simulink model "Manu6DOF_MICO_NE_v6articulation2019b"  (R2019b)
settings: Solver=ode5  StartTime=0.0  StopTime=10.0  FixedStep=0.001  RelTol=1e-3
undefined symbols (not defined in the file): f, Sub02MIHM
libraries: instrumentlib x27, dspnetwork x24, simulink x7, dspmtrx3 x3, dspsrcs4 x1
(part 2 of 3)

== matlab function Manu6DOF_MICO_NE_v6articulation2019b/C1 ==
  data: qm input; C output; dqm input
function C = fcn(qm, dqm)

% theta_1 = qm(1);
% theta_2 = qm(2);
% theta_3 = qm(3);
% theta_4 = qm(4);
% theta_5 = qm(5);
% theta_6 = qm(6);

q1 = qm(1);
q2 = qm(2);
q3 = qm(3);
q4 = qm(4);
q5 = qm(5);
q6 = qm(6);

q1d = dqm(1);
q2d = dqm(2);
q3d = dqm(3);
q4d = dqm(4);
q5d = dqm(5);
q6d = dqm(6);

%%%%%%%%%%%%%%%%%%%%%%%
%function C_c = Cq(q1,q2,q3,q4,q5,q6,q1d,q2d,q3d,q4d,q5d,q6d)
%CQ
%    C_C = CQ(Q1,Q2,Q3,Q4,Q5,Q6,Q1D,Q2D,Q3D,Q4D,Q5D,Q6D)

%    This function was generated by the Symbolic Math Toolbox version 8.4.
%    09-Jul-2020 20:13:25

C = reshape([q1d.*(-2.356599459063229e+4)-q2d.*4.088711718154727e+4+q3d.*2.730577954033007e+5+q4d.*8.285703356363623e+4-q5d.*1.473618543709382e+5+q6d.*7.520537517824024e+4+sqrt(3.0).*q1d.*1.522529520000002e+4+sqrt(3.0).*q2d.*1.015019680000001e+4+sqrt(3.0).*q3d.*3.555581400000001e+4+sqrt(3.0).*q4d.*3.525894120000001e+4+sqrt(3.0).*q5d.*3.780719200000012e+3+sqrt(3.0).*q6d.*2.486339999999987e+3+q1d.*conj(q1).*5.04570275175e+3+q1d.*conj(q2).*4.49975074899e+3+q2d.*conj(q1).*1.49991691633e+3+q1d.*conj(q3).*1.97644016599907e-13+q2d.*conj(q2).*2.99983383266e+3+q3d.*conj(q1).*6.588133886663567e-14+q1d.*conj(q4).*7.944161321388966e-14+q2d.*conj(q3).*1.317626777332713e-13+q3d.*conj(q2).*6.588133886663567e-14+q4d.*conj(q1).*2.648053773796322e-14-q1d.*conj(q5).*7.310773996869955e-14+q2d.*conj(q4).*5.296107547592644e-14+q3d.*conj(q3).*1.07592391394e+3+q4d.*conj(q2).*2.648053773796322e-14-q5d.*conj(q1).*2.436924665623318e-14+q1d.*conj(q6).*2.003216001705283e-13-q2d.*conj(q5).*4.873849331246636e-14+q3d.*conj(q4).*4.3246e+2+q4d.*conj(q3).*4.3246e+2-q5d.*conj(q2).*2.436924665623318e-14+q6d.*conj(q1).*6.677386672350943e-14+q2d.*conj(q6).*1.335477334470189e-13-q3d.*conj(q5).*3.9798e+2+q4d.*conj(q4).*8.6492e+2-q5d.*conj(q3).*3.9798e+2+q6d.*conj(q2).*6.677386672350943e-14+q3d.*conj(q6).*3.635000000000001e+2+q4d.*conj(q5).*3.9798e+2+q5d.*conj(q4).*3.9798e+2+q6d.*conj(q3).*3.635e+2-q4d.*conj(q6).*3.634999999999999e+2+q5d.*conj(q5).*7.9596e+2-q6d.*conj(q4).*3.635e+2-q5d.*conj(q6).*7.269999999999999e+2-q6d.*conj(q5).*7.27e+2+q6d.*conj(q6).*7.270000000000001e+2-sqrt(3.0).*q1d.*conj(q4).*1.29738e+3-sqrt(3.0).*q4d.*conj(q1).*4.3246e+2-sqrt(3.0).*q1d.*conj(q5).*1.19394e+3-sqrt(3.0).*q2d.*conj(q4).*8.6492e+2-sqrt(3.0).*q4d.*conj(q2).*4.3246e+2-sqrt(3.0).*q5d.*conj(q1).*3.9798e+2+sqrt(3.0).*q1d.*conj(q6).*1.0905e+3-sqrt(3.0).*q2d.*conj(q5).*7.9596e+2-sqrt(3.0).*q3d.*conj(q4).*4.3246e+2+sqrt(3.0).*q4d.*conj(q3).*2.902843497617834e-31-sqrt(3.0).*q5d.*conj(q2).*3.9798e+2+sqrt(3.0).*q6d.*conj(q1).*3.635e+2+sqrt(3.0).*q2d.*conj(q6).*7.27e+2-sqrt(3.0).*q3d.*conj(q5).*3.9798e+2-sqrt(3.0).*q4d.*conj(q4).*4.3246e+2+sqrt(3.0).*q5d.*conj(q3).*2.671400025856601e-31+sqrt(3.0).*q6d.*conj(q2).*3.635e+2+sqrt(3.0).*q3d.*conj(q6).*3.635e+2-sqrt(3.0).*q4d.*conj(q5).*3.9798e+2-sqrt(3.0).*q6d.*conj(q3).*4.451591114900629e-14+sqrt(3.0).*q4d.*conj(q6).*3.635e+2-sqrt(3.0).*q5d.*conj(q5).*3.9798e+2-sqrt(3.0).*q6d.*conj(q4).*4.451591114900629e-14+sqrt(3.0).*q5d.*conj(q6).*3.635e+2+sqrt(3.0).*q6d.*conj(q5).*4.879913108190735e-31+sqrt(3.0).*q6d.*conj(q6).*3.635e+2,q1d.*(-4.088711718154727e+4)-q2d.*4.088711718154727e+4+q3d.*1.398366081578192e+5+q4d.*3.824377798181812e+4-q5d.*7.746164638546913e+4+q6d.*4.008902758912012e+4+sqrt(3.0).*q1d.*1.015019680000001e+4+sqrt(3.0).*q2d.*1.015019680000001e+4+sqrt(3.0).*q3d.*3.30182648e+4+sqrt(3.0).*q4d.*3.272139200000001e+4+sqrt(3.0).*q5d.*1.890359600000006e+3+sqrt(3.0).*q6d.*1.243169999999994e+3+q1d.*conj(q1).*1.49991691633e+3+q1d.*conj(q2).*2.99983383266e+3+q2d.*conj(q1).*1.49991691633e+3+q1d.*conj(q3).*1.317626777332713e-13+q2d.*conj(q2).*2.99983383266e+3+q3d.*conj(q1).*3.294066943331783e-14+q1d.*conj(q4).*5.296107547592644e-14+q2d.*conj(q3).*1.317626777332713e-13+q3d.*conj(q2).*6.588133886663567e-14+q4d.*conj(q1).*1.324026886898161e-14-q1d.*conj(q5).*4.873849331246636e-14+q2d.*conj(q4).*5.296107547592644e-14+q3d.*conj(q3).*1.07592391394e+3+q4d.*conj(q2).*2.648053773796322e-14-q5d.*conj(q1).*1.218462332811659e-14+q1d.*conj(q6).*1.335477334470189e-13-q2d.*conj(q5).*4.873849331246636e-14+q3d.*conj(q4).*4.3246e+2+q4d.*conj(q3).*4.3246e+2-q5d.*conj(q2).*2.436924665623318e-14+q6d.*conj(q1).*3.338693336175472e-14+q2d.*conj(q6).*1.335477334470189e-13-q3d.*conj(q5).*3.9798e+2+q4d.*conj(q4).*8.6492e+2-q5d.*conj(q3).*3.9798e+2+q6d.*conj(q2).*6.677386672350943e-14+q3d.*conj(q6).*3.635e+2+q4d.*conj(q5).*3.9798e+2+q5d.*conj(q4).*3.9798e+2+q6d.*conj(q3).*3.635e+2-q4d.*conj(q6).*3.635e+2+q5d.*conj(q5).*7.9596e+2-q6d.*conj(q4).*3.635e+2-q5d.*conj(q6).*7.27e+2-q6d.*conj(q5).*7.27e+2+q6d.*conj(q6).*7.27e+2-sqrt(3.0).*q1d.*conj(q4).*8.6492e+2-sqrt(3.0).*q4d.*conj(q1).*2.1623e+2-sqrt(3.0).*q1d.*conj(q5).*7.9596e+2-sqrt(3.0).*q2d.*conj(q4).*8.6492e+2-sqrt(3.0).*q4d.*conj(q2).*4.3246e+2-sqrt(3.0).*q5d.*conj(q1).*1.9899e+2+sqrt(3.0).*q1d.*conj(q6).*7.27e+2-sqrt(3.0).*q2d.*conj(q5).*7.9596e+2-sqrt(3.0).*q3d.*conj(q4).*2.1623e+2+sqrt(3.0).*q4d.*conj(q3).*2.902843497617834e-31-sqrt(3.0).*q5d.*conj(q2).*3.9798e+2+sqrt(3.0).*q6d.*conj(q1).*1.8175e+2+sqrt(3.0).*q2d.*conj(q6).*7.27e+2-sqrt(3.0).*q3d.*conj(q5).*1.9899e+2-sqrt(3.0).*q4d.*conj(q4).*2.1623e+2+sqrt(3.0).*q5d.*conj(q3).*2.671400025856601e-31+sqrt(3.0).*q6d.*conj(q2).*3.635e+2+sqrt(3.0).*q3d.*conj(q6).*1.8175e+2-sqrt(3.0).*q4d.*conj(q5).*1.9899e+2-sqrt(3.0).*q6d.*conj(q3).*4.451591114900629e-14+sqrt(3.0).*q4d.*conj(q6).*1.8175e+2-sqrt(3.0).*q5d.*conj(q5).*1.9899e+2-sqrt(3.0).*q6d.*conj(q4).*4.451591114900629e-14+sqrt(3.0).*q5d.*conj(q6).*1.8175e+2+sqrt(3.0).*q6d.*conj(q5).*4.879913108190735e-31+sqrt(3.0).*q6d.*conj(q6).*1.8175e+2,q1d.*2.730577954033007e+5+q2d.*1.398366081578192e+5+q3d.*3.095751114833673e+5+q4d.*5.443043298181812e+4-q5d.*6.047936538546912e+4+q6d.*5.627568258912012e+4+sqrt(3.0).*q1d.*3.555581400000001e+4+sqrt(3.0).*q2d.*3.30182648e+4+sqrt(3.0).*q3d.*6.09614312e+4+sqrt(3.0).*q4d.*4.54242006e+4+sqrt(3.0).*q5d.*1.50919214e+4+sqrt(3.0).*q6d.*1.494348499999999e+4+q1d.*conj(q1).*6.588133886663567e-14+q1d.*conj(q2).*6.588133886663567e-14+q2d.*conj(q1).*3.294066943331783e-14+q1d.*conj(q3).*1.07592391394e+3+q2d.*conj(q2).*6.588133886663567e-14+q3d.*conj(q1).*6.588133886663567e-14+q1d.*conj(q4).*4.3246e+2+q2d.*conj(q3).*1.07592391394e+3+q3d.*conj(q2).*6.588133886663567e-14+q4d.*conj(q1).*1.324026886898161e-14-q1d.*conj(q5).*3.9798e+2+q2d.*conj(q4).*4.3246e+2+q3d.*conj(q3).*2.15184782788e+3+q4d.*conj(q2).*1.324026886898161e-14-q5d.*conj(q1).*1.218462332811659e-14+q1d.*conj(q6).*3.635000000000001e+2-q2d.*conj(q5).*3.9798e+2+q3d.*conj(q4).*8.6492e+2+q4d.*conj(q3).*4.3246e+2-q5d.*conj(q2).*1.218462332811659e-14+q6d.*conj(q1).*3.338693336175472e-14+q2d.*conj(q6).*3.635e+2-q3d.*conj(q5).*7.9596e+2+q4d.*conj(q4).*1.08115e+3-q5d.*conj(q3).*3.9798e+2+q6d.*conj(q2).*3.338693336175472e-14+q3d.*conj(q6).*7.27e+2+q4d.*conj(q5).*1.9899e+2+q5d.*conj(q4).*3.9798e+2+q6d.*conj(q3).*3.635e+2-q4d.*conj(q6).*1.8175e+2+q5d.*conj(q5).*5.9697e+2-q6d.*conj(q4).*3.635e+2-q5d.*conj(q6).*5.4525e+2-q6d.*conj(q5).*7.27e+2+q6d.*conj(q6).*9.0875e+2-sqrt(3.0).*q1d.*conj(q4).*4.3246e+2-sqrt(3.0).*q4d.*conj(q1).*2.1623e+2-sqrt(3.0).*q1d.*conj(q5).*3.9798e+2-sqrt(3.0).*q2d.*conj(q4).*2.1623e+2-sqrt(3.0).*q4d.*conj(q2).*2.1623e+2-sqrt(3.0).*q5d.*conj(q1).*1.9899e+2+sqrt(3.0).*q1d.*conj(q6).*3.635e+2-sqrt(3.0).*q2d.*conj(q5).*1.9899e+2+sqrt(3.0).*q3d.*conj(q4).*5.805686995235668e-31+sqrt(3.0).*q4d.*conj(q3).*2.902843497617834e-31-sqrt(3.0).*q5d.*conj(q2).*1.9899e+2+sqrt(3.0).*q6d.*conj(q1).*1.8175e+2+sqrt(3.0).*q2d.*conj(q6).*1.8175e+2+sqrt(3.0).*q3d.*conj(q5).*5.342800051713201e-31+sqrt(3.0).*q4d.*conj(q4).*4.354265246426751e-31+sqrt(3.0).*q5d.*conj(q3).*2.671400025856601e-31+sqrt(3.0).*q6d.*conj(q2).*1.8175e+2-sqrt(3.0).*q3d.*conj(q6).*8.903182229801258e-14+sqrt(3.0).*q4d.*conj(q5).*1.3357000129283e-31-sqrt(3.0).*q6d.*conj(q3).*4.451591114900629e-14-sqrt(3.0).*q4d.*conj(q6).*6.677386672350943e-14-sqrt(3.0).*q5d.*conj(q5).*1.3357000129283e-31-sqrt(3.0).*q6d.*conj(q4).*4.451591114900629e-14-sqrt(3.0).*q5d.*conj(q6).*2.225795557450314e-14+sqrt(3.0).*q6d.*conj(q5).*4.879913108190735e-31-sqrt(3.0).*q6d.*conj(q6).*2.225795557450315e-14,q1d.*8.285703356363623e+4+q2d.*3.824377798181812e+4+q3d.*5.443043298181812e+4+q4d.*1.063745259636362e+5-q5d.*6.426008458546913e+4+q6d.*5.378934258912012e+4+sqrt(3.0).*q1d.*3.525894120000001e+4+sqrt(3.0).*q2d.*3.272139200000001e+4+sqrt(3.0).*q3d.*4.54242006e+4+sqrt(3.0).*q4d.*6.036768560000001e+4+sqrt(3.0).*q5d.*1.50919214e+4+sqrt(3.0).*q6d.*1.494348499999999e+4+q1d.*conj(q1).*2.648053773796322e-14+q1d.*conj(q2).*2.648053773796322e-14+q2d.*conj(q1).*1.324026886898161e-14+q1d.*conj(q3).*4.3246e+2+q2d.*conj(q2).*2.648053773796322e-14+q3d.*conj(q1).*1.324026886898161e-14+q1d.*conj(q4).*8.6492e+2+q2d.*conj(q3).*4.3246e+2+q3d.*conj(q2).*1.324026886898161e-14+q4d.*conj(q1).*2.648053773796322e-14+q1d.*conj(q5).*3.9798e+2+q2d.*conj(q4).*8.6492e+2+q3d.*conj(q3).*4.3246e+2+q4d.*conj(q2).*2.648053773796322e-14-q5d.*conj(q1).*1.218462332811659e-14-q1d.*conj(q6).*3.634999999999999e+2+q2d.*conj(q5).*3.9798e+2+q3d.*conj(q4).*1.08115e+3+q4d.*conj(q3).*4.3246e+2-q5d.*conj(q2).*1.218462332811659e-14+q6d.*conj(q1).*3.338693336175472e-14-q2d.*conj(q6).*3.635e+2+q3d.*conj(q5).*1.9899e+2+q4d.*conj(q4).*1.72984e+3-q5d.*conj(q3).*1.9899e+2+q6d.*conj(q2).*3.338693336175472e-14-q3d.*conj(q6).*1.8175e+2+q4d.*conj(q5).*7.9596e+2+q5d.*conj(q4).*3.9798e+2+q6d.*conj(q3).*1.8175e+2-q4d.*conj(q6).*7.27e+2+q5d.*conj(q5).*9.9495e+2-q6d.*conj(q4).*3.635e+2-q5d.*conj(q6).*9.0875e+2-q6d.*conj(q5).*7.27e+2+q6d.*conj(q6).*5.4525e+2-sqrt(3.0).*q1d.*conj(q1).*4.3246e+2-sqrt(3.0).*q1d.*conj(q2).*4.3246e+2-sqrt(3.0).*q2d.*conj(q1).*2.1623e+2+sqrt(3.0).*q1d.*conj(q3).*2.902843497617834e-31-sqrt(3.0).*q2d.*conj(q2).*4.3246e+2-sqrt(3.0).*q3d.*conj(q1).*2.1623e+2-sqrt(3.0).*q1d.*conj(q4).*4.3246e+2+sqrt(3.0).*q2d.*conj(q3).*2.902843497617834e-31-sqrt(3.0).*q3d.*conj(q2).*2.1623e+2-sqrt(3.0).*q4d.*conj(q1).*4.3246e+2-sqrt(3.0).*q1d.*conj(q5).*3.9798e+2-sqrt(3.0).*q2d.*conj(q4).*2.1623e+2+sqrt(3.0).*q3d.*conj(q3).*2.902843497617834e-31-sqrt(3.0).*q4d.*conj(q2).*4.3246e+2-sqrt(3.0).*q5d.*conj(q1).*1.9899e+2+sqrt(3.0).*q1d.*conj(q6).*3.635e+2-sqrt(3.0).*q2d.*conj(q5).*1.9899e+2+sqrt(3.0).*q3d.*conj(q4).*4.354265246426751e-31+sqrt(3.0).*q4d.*conj(q3).*2.902843497617834e-31-sqrt(3.0).*q5d.*conj(q2).*1.9899e+2+sqrt(3.0).*q6d.*conj(q1).*1.8175e+2+sqrt(3.0).*q2d.*conj(q6).*1.8175e+2+sqrt(3.0).*q3d.*conj(q5).*1.3357000129283e-31+sqrt(3.0).*q4d.*conj(q4).*5.805686995235668e-31+sqrt(3.0).*q5d.*conj(q3).*1.3357000129283e-31+sqrt(3.0).*q6d.*conj(q2).*1.8175e+2-sqrt(3.0).*q3d.*conj(q6).*6.677386672350943e-14-sqrt(3.0).*q6d.*conj(q3).*2.225795557450315e-14-sqrt(3.0).*q4d.*conj(q6).*8.903182229801258e-14-sqrt(3.0).*q5d.*conj(q5).*2.671400025856601e-31-sqrt(3.0).*q6d.*conj(q4).*4.451591114900629e-14-sqrt(3.0).*q5d.*conj(q6).*2.225795557450314e-14+sqrt(3.0).*q6d.*conj(q5).*4.879913108190735e-31-sqrt(3.0).*q6d.*conj(q6).*2.225795557450315e-14,q1d.*(-1.473618543709382e+5)-q2d.*7.746164638546913e+4-q3d.*6.047936538546912e+4-q4d.*6.426008458546913e+4-q5d.*1.247394499709383e+5+q6d.*5.254617258912011e+4+sqrt(3.0).*q1d.*3.780719200000012e+3+sqrt(3.0).*q2d.*1.890359600000006e+3+sqrt(3.0).*q3d.*1.50919214e+4+sqrt(3.0).*q4d.*1.50919214e+4+sqrt(3.0).*q5d.*6.381198636905707e-12-sqrt(3.0).*q6d.*9.113935495870542e-12-q1d.*conj(q1).*2.436924665623318e-14-q1d.*conj(q2).*2.436924665623318e-14-q2d.*conj(q1).*1.218462332811659e-14-q1d.*conj(q3).*3.9798e+2-q2d.*conj(q2).*2.436924665623318e-14-q3d.*conj(q1).*1.218462332811659e-14+q1d.*conj(q4).*3.9798e+2-q2d.*conj(q3).*3.9798e+2-q3d.*conj(q2).*1.218462332811659e-14-q4d.*conj(q1).*1.218462332811659e-14+q1d.*conj(q5).*7.9596e+2+q2d.*conj(q4).*3.9798e+2-q3d.*conj(q3).*3.9798e+2-q4d.*conj(q2).*1.218462332811659e-14-q5d.*conj(q1).*2.436924665623318e-14-q1d.*conj(q6).*7.269999999999999e+2+q2d.*conj(q5).*7.9596e+2+q3d.*conj(q4).*3.9798e+2-q4d.*conj(q3).*1.9899e+2-q5d.*conj(q2).*2.436924665623318e-14+q6d.*conj(q1).*3.338693336175472e-14-q2d.*conj(q6).*7.27e+2+q3d.*conj(q5).*5.9697e+2+q4d.*conj(q4).*3.9798e+2-q5d.*conj(q3).*3.9798e+2+q6d.*conj(q2).*3.338693336175472e-14-q3d.*conj(q6).*5.4525e+2+q4d.*conj(q5).*9.9495e+2+q5d.*conj(q4).*3.9798e+2+q6d.*conj(q3).*1.8175e+2-q4d.*conj(q6).*9.0875e+2+q5d.*conj(q5).*1.59192e+3-q6d.*conj(q4).*1.8175e+2-q5d.*conj(q6).*1.454e+3-q6d.*conj(q5).*7.27e+2+q6d.*conj(q6).*3.635e+2-sqrt(3.0).*q1d.*conj(q1).*3.9798e+2-sqrt(3.0).*q1d.*conj(q2).*3.9798e+2-sqrt(3.0).*q2d.*conj(q1).*1.9899e+2+sqrt(3.0).*q1d.*conj(q3).*2.671400025856601e-31-sqrt(3.0).*q2d.*conj(q2).*3.9798e+2-sqrt(3.0).*q3d.*conj(q1).*1.9899e+2+sqrt(3.0).*q2d.*conj(q3).*2.671400025856601e-31-sqrt(3.0).*q3d.*conj(q2).*1.9899e+2-sqrt(3.0).*q4d.*conj(q1).*1.9899e+2-sqrt(3.0).*q1d.*conj(q5).*3.9798e+2+sqrt(3.0).*q3d.*conj(q3).*2.671400025856601e-31-sqrt(3.0).*q4d.*conj(q2).*1.9899e+2-sqrt(3.0).*q5d.*conj(q1).*3.9798e+2+sqrt(3.0).*q1d.*conj(q6).*3.635e+2-sqrt(3.0).*q2d.*conj(q5).*1.9899e+2+sqrt(3.0).*q4d.*conj(q3).*1.3357000129283e-31-sqrt(3.0).*q5d.*conj(q2).*3.9798e+2+sqrt(3.0).*q6d.*conj(q1).*1.8175e+2+sqrt(3.0).*q2d.*conj(q6).*1.8175e+2-sqrt(3.0).*q3d.*conj(q5).*1.3357000129283e-31+sqrt(3.0).*q5d.*conj(q3).*2.671400025856601e-31+sqrt(3.0).*q6d.*conj(q2).*1.8175e+2-sqrt(3.0).*q3d.*conj(q6).*2.225795557450314e-14-sqrt(3.0).*q4d.*conj(q5).*2.671400025856601e-31-sqrt(3.0).*q6d.*conj(q3).*2.225795557450315e-14-sqrt(3.0).*q4d.*conj(q6).*2.225795557450314e-14-sqrt(3.0).*q5d.*conj(q5).*5.342800051713201e-31-sqrt(3.0).*q6d.*conj(q4).*2.225795557450314e-14+sqrt(3.0).*q5d.*conj(q6).*9.75982621638147e-31+sqrt(3.0).*q6d.*conj(q5).*4.879913108190735e-31-sqrt(3.0).*q6d.*conj(q6).*4.879913108190735e-31,q1d.*7.520537517824024e+4+q2d.*4.008902758912012e+4+q3d.*5.627568258912012e+4+q4d.*5.378934258912012e+4+q5d.*5.254617258912011e+4+q6d.*1.100650251782402e+5+sqrt(3.0).*q1d.*2.486339999999987e+3+sqrt(3.0).*q2d.*1.243169999999994e+3+sqrt(3.0).*q3d.*1.494348499999999e+4+sqrt(3.0).*q4d.*1.494348499999999e+4-sqrt(3.0).*q5d.*9.113935495870542e-12-sqrt(3.0).*q6d.*1.806405785964667e-11+q1d.*conj(q1).*6.677386672350943e-14+q1d.*conj(q2).*6.677386672350943e-14+q2d.*conj(q1).*3.338693336175472e-14+q1d.*conj(q3).*3.635e+2+q2d.*conj(q2).*6.677386672350943e-14+q3d.*conj(q1).*3.338693336175472e-14-q1d.*conj(q4).*3.635e+2+q2d.*conj(q3).*3.635e+2+q3d.*conj(q2).*3.338693336175472e-14+q4d.*conj(q1).*3.338693336175472e-14-q1d.*conj(q5).*7.27e+2-q2d.*conj(q4).*3.635e+2+q3d.*conj(q3).*3.635e+2+q4d.*conj(q2).*3.338693336175472e-14+q5d.*conj(q1).*3.338693336175472e-14+q1d.*conj(q6).*7.270000000000001e+2-q2d.*conj(q5).*7.27e+2-q3d.*conj(q4).*3.635e+2+q4d.*conj(q3).*1.8175e+2+q5d.*conj(q2).*3.338693336175472e-14+q6d.*conj(q1).*6.677386672350943e-14+q2d.*conj(q6).*7.27e+2-q3d.*conj(q5).*7.27e+2-q4d.*conj(q4).*3.635e+2+q5d.*conj(q3).*1.8175e+2+q6d.*conj(q2).*6.677386672350943e-14+q3d.*conj(q6).*9.0875e+2-q4d.*conj(q5).*7.27e+2-q5d.*conj(q4).*1.8175e+2+q6d.*conj(q3).*3.635e+2+q4d.*conj(q6).*5.4525e+2-q5d.*conj(q5).*7.27e+2-q6d.*conj(q4).*3.635e+2+q5d.*conj(q6).*3.635e+2-q6d.*conj(q5).*7.27e+2+q6d.*conj(q6).*1.454e+3+sqrt(3.0).*q1d.*conj(q1).*3.635e+2+sqrt(3.0).*q1d.*conj(q2).*3.635e+2+sqrt(3.0).*q2d.*conj(q1).*1.8175e+2-sqrt(3.0).*q1d.*conj(q3).*4.451591114900629e-14+sqrt(3.0).*q2d.*conj(q2).*3.635e+2+sqrt(3.0).*q3d.*conj(q1).*1.8175e+2-sqrt(3.0).*q1d.*conj(q4).*4.451591114900629e-14-sqrt(3.0).*q2d.*conj(q3).*4.451591114900629e-14+sqrt(3.0).*q3d.*conj(q2).*1.8175e+2+sqrt(3.0).*q4d.*conj(q1).*1.8175e+2+sqrt(3.0).*q1d.*conj(q5).*4.879913108190735e-31-sqrt(3.0).*q2d.*conj(q4).*4.451591114900629e-14-sqrt(3.0).*q3d.*conj(q3).*4.451591114900629e-14+sqrt(3.0).*q4d.*conj(q2).*1.8175e+2+sqrt(3.0).*q5d.*conj(q1).*1.8175e+2+sqrt(3.0).*q1d.*conj(q6).*3.635e+2+sqrt(3.0).*q2d.*conj(q5).*4.879913108190735e-31-sqrt(3.0).*q3d.*conj(q4).*4.451591114900629e-14-sqrt(3.0).*q4d.*conj(q3).*2.225795557450315e-14+sqrt(3.0).*q5d.*conj(q2).*1.8175e+2+sqrt(3.0).*q6d.*conj(q1).*3.635e+2+sqrt(3.0).*q2d.*conj(q6).*1.8175e+2+sqrt(3.0).*q3d.*conj(q5).*4.879913108190735e-31-sqrt(3.0).*q4d.*conj(q4).*4.451591114900629e-14-sqrt(3.0).*q5d.*conj(q3).*2.225795557450315e-14+sqrt(3.0).*q6d.*conj(q2).*3.635e+2-sqrt(3.0).*q3d.*conj(q6).*2.225795557450315e-14+sqrt(3.0).*q4d.*conj(q5).*4.879913108190735e-31-sqrt(3.0).*q5d.*conj(q4).*2.225795557450314e-14-sqrt(3.0).*q6d.*conj(q3).*4.451591114900629e-14-sqrt(3.0).*q4d.*conj(q6).*2.225795557450315e-14+sqrt(3.0).*q5d.*conj(q5).*4.879913108190735e-31-sqrt(3.0).*q6d.*conj(q4).*4.451591114900629e-14-sqrt(3.0).*q5d.*conj(q6).*4.879913108190735e-31+sqrt(3.0).*q6d.*conj(q5).*4.879913108190735e-31-sqrt(3.0).*q6d.*conj(q6).*1.46397393245722e-30,q1d.*(-4.088711718154727e+4)-q2d.*4.088711718154727e+4+q3d.*1.398366081578192e+5+q4d.*3.824377798181812e+4-q5d.*7.746164638546913e+4+q6d.*4.008902758912012e+4+sqrt(3.0).*q1d.*1.015019680000001e+4+sqrt(3.0).*q2d.*1.015019680000001e+4+sqrt(3.0).*q3d.*3.30182648e+4+sqrt(3.0).*q4d.*3.272139200000001e+4+sqrt(3.0).*q5d.*1.890359600000006e+3+sqrt(3.0).*q6d.*1.243169999999994e+3+q1d.*conj(q1).*1.49991691633e+3+q1d.*conj(q2).*2.99983383266e+3+q2d.*conj(q1).*1.49991691633e+3+q1d.*conj(q3).*1.317626777332713e-13+q2d.*conj(q2).*2.99983383266e+3+q3d.*conj(q1).*3.294066943331783e-14+q1d.*conj(q4).*5.296107547592644e-14+q2d.*conj(q3).*1.317626777332713e-13+q3d.*conj(q2).*6.588133886663567e-14+q4d.*conj(q1).*1.324026886898161e-14-q1d.*conj(q5).*4.873849331246636e-14+q2d.*conj(q4).*5.296107547592644e-14+q3d.*conj(q3).*1.07592391394e+3+q4d.*conj(q2).*2.648053773796322e-14-q5d.*conj(q1).*1.218462332811659e-14+q1d.*conj(q6).*1.335477334470189e-13-q2d.*conj(q5).*4.873849331246636e-14+q3d.*conj(q4).*4.3246e+2+q4d.*conj(q3).*4.3246e+2-q5d.*conj(q2).*2.436924665623318e-14+q6d.*conj(q1).*3.338693336175472e-14+q2d.*conj(q6).*1.335477334470189e-13-q3d.*conj(q5).*3.9798e+2+q4d.*conj(q4).*8.6492e+2-q5d.*conj(q3).*3.9798e+2+q6d.*conj(q2).*6.677386672350943e-14+q3d.*conj(q6).*3.635e+2+q4d.*conj(q5).*3.9798e+2+q5d.*conj(q4).*3.9798e+2+q6d.*conj(q3).*3.635e+2-q4d.*conj(q6).*3.635e+2+q5d.*conj(q5).*7.9596e+2-q6d.*conj(q4).*3.635e+2-q5d.*conj(q6).*7.27e+2-q6d.*conj(q5).*7.27e+2+q6d.*conj(q6).*7.27e+2-sqrt(3.0).*q1d.*conj(q4).*8.6492e+2-sqrt(3.0).*q4d.*conj(q1).*2.1623e+2-sqrt(3.0).*q1d.*conj(q5).*7.9596e+2-sqrt(3.0).*q2d.*conj(q4).*8.6492e+2-sqrt(3.0).*q4d.*conj(q2).*4.3246e+2-sqrt(3.0).*q5d.*conj(q1).*1.9899e+2+sqrt(3.0).*q1d.*conj(q6).*7.27e+2-sqrt(3.0).*q2d.*conj(q5).*7.9596e+2-sqrt(3.0).*q3d.*conj(q4).*2.1623e+2+sqrt(3.0).*q4d.*conj(q3).*2.902843497617834e-31-sqrt(3.0).*q5d.*conj(q2).*3.9798e+2+sqrt(3.0).*q6d.*conj(q1).*1.8175e+2+sqrt(3.0).*q2d.*conj(q6).*7.27e+2-sqrt(3.0).*q3d.*conj(q5).*1.9899e+2-sqrt(3.0).*q4d.*conj(q4).*2.1623e+2+sqrt(3.0).*q5d.*conj(q3).*2.671400025856601e-31+sqrt(3.0).*q6d.*conj(q2).*3.635e+2+sqrt(3.0).*q3d.*conj(q6).*1.8175e+2-sqrt(3.0).*q4d.*conj(q5).*1.9899e+2-sqrt(3.0).*q6d.*conj(q3).*4.451591114900629e-14+sqrt(3.0).*q4d.*conj(q6).*1.8175e+2-sqrt(3.0).*q5d.*conj(q5).*1.9899e+2-sqrt(3.0).*q6d.*conj(q4).*4.451591114900629e-14+sqrt(3.0).*q5d.*conj(q6).*1.8175e+2+sqrt(3.0).*q6d.*conj(q5).*4.879913108190735e-31+sqrt(3.0).*q6d.*conj(q6).*1.8175e+2,q1d.*(-4.088711718154727e+4)-q2d.*6.13306757723209e+4-q3d.*2.328647425539134e+4-q4d.*3.62564476e+4-q5d.*3.774528120000001e+4-q6d.*2.491429e+4+sqrt(3.0).*q1d.*1.015019680000001e+4+sqrt(3.0).*q2d.*1.522529520000002e+4+sqrt(3.0).*q3d.*3.555581400000001e+4+sqrt(3.0).*q4d.*3.525894120000001e+4+sqrt(3.0).*q5d.*3.780719200000005e+3+sqrt(3.0).*q6d.*2.486340000000006e+3+q1d.*conj(q1).*1.49991691633e+3+q1d.*conj(q2).*2.99983383266e+3+q1d.*conj(q3).*1.317626777332713e-13+q2d.*conj(q2).*4.49975074899e+3+q1d.*conj(q4).*5.296107547592644e-14+q2d.*conj(q3).*1.97644016599907e-13+q3d.*conj(q2).*6.588133886663567e-14-q1d.*conj(q5).*4.873849331246636e-14+q2d.*conj(q4).*7.944161321388966e-14+q3d.*conj(q3).*1.07592391394e+3+q4d.*conj(q2).*2.648053773796322e-14+q1d.*conj(q6).*1.335477334470189e-13-q2d.*conj(q5).*7.310773996869955e-14+q3d.*conj(q4).*4.3246e+2+q4d.*conj(q3).*4.3246e+2-q5d.*conj(q2).*2.436924665623318e-14+q2d.*conj(q6).*2.003216001705283e-13-q3d.*conj(q5).*3.9798e+2+q4d.*conj(q4).*8.6492e+2-q5d.*conj(q3).*3.9798e+2+q6d.*conj(q2).*6.677386672350943e-14+q3d.*conj(q6).*3.635000000000001e+2+q4d.*conj(q5).*3.9798e+2+q5d.*conj(q4).*3.9798e+2+q6d.*conj(q3).*3.635e+2-q4d.*conj(q6).*3.634999999999999e+2+q5d.*conj(q5).*7.9596e+2-q6d.*conj(q4).*3.635e+2-q5d.*conj(q6).*7.269999999999999e+2-q6d.*conj(q5).*7.27e+2+q6d.*conj(q6).*7.270000000000001e+2-sqrt(3.0).*q1d.*conj(q4).*8.6492e+2-sqrt(3.0).*q1d.*conj(q5).*7.9596e+2-sqrt(3.0).*q2d.*conj(q4).*1.29738e+3-sqrt(3.0).*q4d.*conj(q2).*4.3246e+2+sqrt(3.0).*q1d.*conj(q6).*7.27e+2-sqrt(3.0).*q2d.*conj(q5).*1.19394e+3-sqrt(3.0).*q3d.*conj(q4).*4.3246e+2+sqrt(3.0).*q4d.*conj(q3).*2.902843497617834e-31-sqrt(3.0).*q5d.*conj(q2).*3.9798e+2+sqrt(3.0).*q2d.*conj(q6).*1.0905e+3-sqrt(3.0).*q3d.*conj(q5).*3.9798e+2-sqrt(3.0).*q4d.*conj(q4).*4.3246e+2+sqrt(3.0).*q5d.*conj(q3).*2.671400025856601e-31+sqrt(3.0).*q6d.*conj(q2).*3.635e+2+sqrt(3.0).*q3d.*conj(q6).*3.635e+2-sqrt(3.0).*q4d.*conj(q5).*3.9798e+2-sqrt(3.0).*q6d.*conj(q3).*4.451591114900629e-14+sqrt(3.0).*q4d.*conj(q6).*3.635e+2-sqrt(3.0).*q5d.*conj(q5).*3.9798e+2-sqrt(3.0).*q6d.*conj(q4).*4.451591114900629e-14+sqrt(3.0).*q5d.*conj(q6).*3.635e+2+sqrt(3.0).*q6d.*conj(q5).*4.879913108190735e-31+sqrt(3.0).*q6d.*conj(q6).*3.635e+2,q1d.*1.398366081578192e+5-q2d.*2.328647425539134e+4+q3d.*1.323084182467521e+4-q4d.*5.126307600000002e+3-q5d.*5.671078800000006e+3+q6d.*6.215850000000002e+3+sqrt(3.0).*q1d.*3.30182648e+4+sqrt(3.0).*q2d.*3.555581400000001e+4+sqrt(3.0).*q3d.*6.09614312e+4+sqrt(3.0).*q4d.*4.54242006e+4+sqrt(3.0).*q5d.*1.50919214e+4+sqrt(3.0).*q6d.*1.4943485e+4+q1d.*conj(q1).*3.294066943331783e-14+q1d.*conj(q2).*6.588133886663567e-14+q1d.*conj(q3).*1.07592391394e+3+q2d.*conj(q2).*6.588133886663567e-14+q1d.*conj(q4).*4.3246e+2+q2d.*conj(q3).*1.07592391394e+3+q3d.*conj(q2).*6.588133886663567e-14-q1d.*conj(q5).*3.9798e+2+q2d.*conj(q4).*4.3246e+2+q3d.*conj(q3).*2.15184782788e+3+q4d.*conj(q2).*1.324026886898161e-14+q1d.*conj(q6).*3.635e+2-q2d.*conj(q5).*3.9798e+2+q3d.*conj(q4).*8.6492e+2+q4d.*conj(q3).*4.3246e+2-q5d.*conj(q2).*1.218462332811659e-14+q2d.*conj(q6).*3.635000000000001e+2-q3d.*conj(q5).*7.9596e+2+q4d.*conj(q4).*1.08115e+3-q5d.*conj(q3).*3.9798e+2+q6d.*conj(q2).*3.338693336175472e-14+q3d.*conj(q6).*7.27e+2+q4d.*conj(q5).*1.9899e+2+q5d.*conj(q4).*3.9798e+2+q6d.*conj(q3).*3.635e+2-q4d.*conj(q6).*1.8175e+2+q5d.*conj(q5).*5.9697e+2-q6d.*conj(q4).*3.635e+2-q5d.*conj(q6).*5.4525e+2-q6d.*conj(q5).*7.27e+2+q6d.*conj(q6).*9.0875e+2-sqrt(3.0).*q1d.*conj(q4).*2.1623e+2-sqrt(3.0).*q1d.*conj(q5).*1.9899e+2-sqrt(3.0).*q2d.*conj(q4).*4.3246e+2-sqrt(3.0).*q4d.*conj(q2).*2.1623e+2+sqrt(3.0).*q1d.*conj(q6).*1.8175e+2-sqrt(3.0).*q2d.*conj(q5).*3.9798e+2+sqrt(3.0).*q3d.*conj(q4).*5.805686995235668e-31+sqrt(3.0).*q4d.*conj(q3).*2.902843497617834e-31-sqrt(3.0).*q5d.*conj(q2).*1.9899e+2+sqrt(3.0).*q2d.*conj(q6).*3.635e+2+sqrt(3.0).*q3d.*conj(q5).*5.342800051713201e-31+sqrt(3.0).*q4d.*conj(q4).*4.354265246426751e-31+sqrt(3.0).*q5d.*conj(q3).*2.671400025856601e-31+sqrt(3.0).*q6d.*conj(q2).*1.8175e+2-sqrt(3.0).*q3d.*conj(q6).*8.903182229801258e-14+sqrt(3.0).*q4d.*conj(q5).*1.3357000129283e-31-sqrt(3.0).*q6d.*conj(q3).*4.451591114900629e-14-sqrt(3.0).*q4d.*conj(q6).*6.677386672350943e-14-sqrt(3.0).*q5d.*conj(q5).*1.3357000129283e-31-sqrt(3.0).*q6d.*conj(q4).*4.451591114900629e-14-sqrt(3.0).*q5d.*conj(q6).*2.225795557450314e-14+sqrt(3.0).*q6d.*conj(q5).*4.879913108190735e-31-sqrt(3.0).*q6d.*conj(q6).*2.225795557450315e-14,q1d.*3.824377798181812e+4-q2d.*3.62564476e+4-q3d.*5.126307600000002e+3-q4d.*1.273895520000001e+4-q5d.*9.451798000000009e+3+q6d.*3.729509999999998e+3+sqrt(3.0).*q1d.*3.272139200000001e+4+sqrt(3.0).*q2d.*3.525894120000001e+4+sqrt(3.0).*q3d.*4.54242006e+4+sqrt(3.0).*q4d.*6.03676856e+4+sqrt(3.0).*q5d.*1.50919214e+4+sqrt(3.0).*q6d.*1.4943485e+4+q1d.*conj(q1).*1.324026886898161e-14+q1d.*conj(q2).*2.648053773796322e-14+q1d.*conj(q3).*4.3246e+2+q2d.*conj(q2).*2.648053773796322e-14+q1d.*conj(q4).*8.6492e+2+q2d.*conj(q3).*4.3246e+2+q3d.*conj(q2).*1.324026886898161e-14+q1d.*conj(q5).*3.9798e+2+q2d.*conj(q4).*8.6492e+2+q3d.*conj(q3).*4.3246e+2+q4d.*conj(q2).*2.648053773796322e-14-q1d.*conj(q6).*3.635e+2+q2d.*conj(q5).*3.9798e+2+q3d.*conj(q4).*1.08115e+3+q4d.*conj(q3).*4.3246e+2-q5d.*conj(q2).*1.218462332811659e-14-q2d.*conj(q6).*3.634999999999999e+2+q3d.*conj(q5).*1.9899e+2+q4d.*conj(q4).*1.72984e+3-q5d.*conj(q3).*1.9899e+2+q6d.*conj(q2).*3.338693336175472e-14-q3d.*conj(q6).*1.8175e+2+q4d.*conj(q5).*7.9596e+2+q5d.*conj(q4).*3.9798e+2+q6d.*conj(q3).*1.8175e+2-q4d.*conj(q6).*7.27e+2+q5d.*conj(q5).*9.9495e+2-q6d.*conj(q4).*3.635e+2-q5d.*conj(q6).*9.0875e+2-q6d.*conj(q5).*7.27e+2+q6d.*conj(q6).*5.4525e+2-sqrt(3.0).*q1d.*conj(q1).*2.1623e+2-sqrt(3.0).*q1d.*conj(q2).*4.3246e+2+sqrt(3.0).*q1d.*conj(q3).*2.902843497617834e-31-sqrt(3.0).*q2d.*conj(q2).*4.3246e+2-sqrt(3.0).*q1d.*conj(q4).*2.1623e+2+sqrt(3.0).*q2d.*conj(q3).*2.902843497617834e-31-sqrt(3.0).*q3d.*conj(q2).*2.1623e+2-sqrt(3.0).*q1d.*conj(q5).*1.9899e+2-sqrt(3.0).*q2d.*conj(q4).*4.3246e+2+sqrt(3.0).*q3d.*conj(q3).*2.902843497617834e-31-sqrt(3.0).*q4d.*conj(q2).*4.3246e+2+sqrt(3.0).*q1d.*conj(q6).*1.8175e+2-sqrt(3.0).*q2d.*conj(q5).*3.9798e+2+sqrt(3.0).*q3d.*conj(q4).*4.354265246426751e-31+sqrt(3.0).*q4d.*conj(q3).*2.902843497617834e-31-sqrt(3.0).*q5d.*conj(q2).*1.9899e+2+sqrt(3.0).*q2d.*conj(q6).*3.635e+2+sqrt(3.0).*q3d.*conj(q5).*1.3357000129283e-31+sqrt(3.0).*q4d.*conj(q4).*5.805686995235668e-31+sqrt(3.0).*q5d.*conj(q3).*1.3357000129283e-31+sqrt(3.0).*q6d.*conj(q2).*1.8175e+2-sqrt(3.0).*q3d.*conj(q6).*6.677386672350943e-14-sqrt(3.0).*q6d.*conj(q3).*2.225795557450315e-14-sqrt(3.0).*q4d.*conj(q6).*8.903182229801258e-14-sqrt(3.0).*q5d.*conj(q5).*2.671400025856601e-31-sqrt(3.0).*q6d.*conj(q4).*4.451591114900629e-14-sqrt(3.0).*q5d.*conj(q6).*2.225795557450314e-14+sqrt(3.0).*q6d.*conj(q5).*4.879913108190735e-31-sqrt(3.0).*q6d.*conj(q6).*2.225795557450315e-14,q1d.*(-7.746164638546913e+4)-q2d.*3.774528120000001e+4-q3d.*5.671078800000006e+3-q4d.*9.451798000000009e+3-q5d.*1.512287680000001e+4+q6d.*2.486339999999996e+3+sqrt(3.0).*q1d.*1.890359600000006e+3+sqrt(3.0).*q2d.*3.780719200000005e+3+sqrt(3.0).*q3d.*1.50919214e+4+sqrt(3.0).*q4d.*1.50919214e+4-sqrt(3.0).*q5d.*3.308806364588508e-13+sqrt(3.0).*q6d.*8.190656604720473e-14-q1d.*conj(q1).*1.218462332811659e-14-q1d.*conj(q2).*2.436924665623318e-14-q1d.*conj(q3).*3.9798e+2-q2d.*conj(q2).*2.436924665623318e-14+q1d.*conj(q4).*3.9798e+2-q2d.*conj(q3).*3.9798e+2-q3d.*conj(q2).*1.218462332811659e-14+q1d.*conj(q5).*7.9596e+2+q2d.*conj(q4).*3.9798e+2-q3d.*conj(q3).*3.9798e+2-q4d.*conj(q2).*1.218462332811659e-14-q1d.*conj(q6).*7.27e+2+q2d.*conj(q5).*7.9596e+2+q3d.*conj(q4).*3.9798e+2-q4d.*conj(q3).*1.9899e+2-q5d.*conj(q2).*2.436924665623318e-14-q2d.*conj(q6).*7.269999999999999e+2+q3d.*conj(q5).*5.9697e+2+q4d.*conj(q4).*3.9798e+2-q5d.*conj(q3).*3.9798e+2+q6d.*conj(q2).*3.338693336175472e-14-q3d.*conj(q6).*5.4525e+2+q4d.*conj(q5).*9.9495e+2+q5d.*conj(q4).*3.9798e+2+q6d.*conj(q3).*1.8175e+2-q4d.*conj(q6).*9.0875e+2+q5d.*conj(q5).*1.59192e+3-q6d.*conj(q4).*1.8175e+2-q5d.*conj(q6).*1.454e+3-q6d.*conj(q5).*7.27e+2+q6d.*conj(q6).*3.635e+2-sqrt(3.0).*q1d.*conj(q1).*1.9899e+2-sqrt(3.0).*q1d.*conj(q2).*3.9798e+2+sqrt(3.0).*q1d.*conj(q3).*2.671400025856601e-31-sqrt(3.0).*q2d.*conj(q2).*3.9798e+2+sqrt(3.0).*q2d.*conj(q3).*2.671400025856601e-31-sqrt(3.0).*q3d.*conj(q2).*1.9899e+2-sqrt(3.0).*q1d.*conj(q5).*1.9899e+2+sqrt(3.0).*q3d.*conj(q3).*2.671400025856601e-31-sqrt(3.0).*q4d.*conj(q2).*1.9899e+2+sqrt(3.0).*q1d.*conj(q6).*1.8175e+2-sqrt(3.0).*q2d.*conj(q5).*3.9798e+2+sqrt(3.0).*q4d.*conj(q3).*1.3357000129283e-31-sqrt(3.0).*q5d.*conj(q2).*3.9798e+2+sqrt(3.0).*q2d.*conj(q6).*3.635e+2-sqrt(3.0).*q3d.*conj(q5).*1.3357000129283e-31+sqrt(3.0).*q5d.*conj(q3).*2.671400025856601e-31+sqrt(3.0).*q6d.*conj(q2).*1.8175e+2-sqrt(3.0).*q3d.*conj(q6).*2.225795557450314e-14-sqrt(3.0).*q4d.*conj(q5).*2.671400025856601e-31-sqrt(3.0).*q6d.*conj(q3).*2.225795557450315e-14-sqrt(3.0).*q4d.*conj(q6).*2.225795557450314e-14-sqrt(3.0).*q5d.*conj(q5).*5.342800051713201e-31-sqrt(3.0).*q6d.*conj(q4).*2.225795557450314e-14+sqrt(3.0).*q5d.*conj(q6).*9.75982621638147e-31+sqrt(3.0).*q6d.*conj(q5).*4.879913108190735e-31-sqrt(3.0).*q6d.*conj(q6).*4.879913108190735e-31,q1d.*4.008902758912012e+4-q2d.*2.491429e+4+q3d.*6.215850000000002e+3+q4d.*3.729509999999998e+3+q5d.*2.486339999999996e+3+q6d.*9.94536e+3+sqrt(3.0).*q1d.*1.243169999999994e+3+sqrt(3.0).*q2d.*2.486340000000006e+3+sqrt(3.0).*q3d.*1.4943485e+4+sqrt(3.0).*q4d.*1.4943485e+4+sqrt(3.0).*q5d.*8.190656604720473e-14+sqrt(3.0).*q6d.*3.276262641888189e-13+q1d.*conj(q1).*3.338693336175472e-14+q1d.*conj(q2).*6.677386672350943e-14+q1d.*conj(q3).*3.635e+2+q2d.*conj(q2).*6.677386672350943e-14-q1d.*conj(q4).*3.635e+2+q2d.*conj(q3).*3.635e+2+q3d.*conj(q2).*3.338693336175472e-14-q1d.*conj(q5).*7.27e+2-q2d.*conj(q4).*3.635e+2+q3d.*conj(q3).*3.635e+2+q4d.*conj(q2).*3.338693336175472e-14+q1d.*conj(q6).*7.27e+2-q2d.*conj(q5).*7.27e+2-q3d.*conj(q4).*3.635e+2+q4d.*conj(q3).*1.8175e+2+q5d.*conj(q2).*3.338693336175472e-14+q2d.*conj(q6).*7.270000000000001e+2-q3d.*conj(q5).*7.27e+2-q4d.*conj(q4).*3.635e+2+q5d.*conj(q3).*1.8175e+2+q6d.*conj(q2).*6.677386672350943e-14+q3d.*conj(q6).*9.0875e+2-q4d.*conj(q5).*7.27e+2-q5d.*conj(q4).*1.8175e+2+q6d.*conj(q3).*3.635e+2+q4d.*conj(q6).*5.4525e+2-q5d.*conj(q5).*7.27e+2-q6d.*conj(q4).*3.635e+2+q5d.*conj(q6).*3.635e+2-q6d.*conj(q5).*7.27e+2+q6d.*conj(q6).*1.454e+3+sqrt(3.0).*q1d.*conj(q1).*1.8175e+2+sqrt(3.0).*q1d.*conj(q2).*3.635e+2-sqrt(3.0).*q1d.*conj(q3).*4.451591114900629e-14+sqrt(3.0).*q2d.*conj(q2).*3.635e+2-sqrt(3.0).*q1d.*conj(q4).*4.451591114900629e-14-sqrt(3.0).*q2d.*conj(q3).*4.451591114900629e-14+sqrt(3.0).*q3d.*conj(q2).*1.8175e+2+sqrt(3.0).*q1d.*conj(q5).*4.879913108190735e-31-sqrt(3.0).*q2d.*conj(q4).*4.451591114900629e-14-sqrt(3.0).*q3d.*conj(q3).*4.451591114900629e-14+sqrt(3.0).*q4d.*conj(q2).*1.8175e+2+sqrt(3.0).*q1d.*conj(q6).*1.8175e+2+sqrt(3.0).*q2d.*conj(q5).*4.879913108190735e-31-sqrt(3.0).*q3d.*conj(q4).*4.451591114900629e-14-sqrt(3.0).*q4d.*conj(q3).*2.225795557450315e-14+sqrt(3.0).*q5d.*conj(q2).*1.8175e+2+sqrt(3.0).*q2d.*conj(q6).*3.635e+2+sqrt(3.0).*q3d.*conj(q5).*4.879913108190735e-31-sqrt(3.0).*q4d.*conj(q4).*4.451591114900629e-14-sqrt(3.0).*q5d.*conj(q3).*2.225795557450315e-14+sqrt(3.0).*q6d.*conj(q2).*3.635e+2-sqrt(3.0).*q3d.*conj(q6).*2.225795557450315e-14+sqrt(3.0).*q4d.*conj(q5).*4.879913108190735e-31-sqrt(3.0).*q5d.*conj(q4).*2.225795557450314e-14-sqrt(3.0).*q6d.*conj(q3).*4.451591114900629e-14-sqrt(3.0).*q4d.*conj(q6).*2.225795557450315e-14+sqrt(3.0).*q5d.*conj(q5).*4.879913108190735e-31-sqrt(3.0).*q6d.*conj(q4).*4.451591114900629e-14-sqrt(3.0).*q5d.*conj(q6).*4.879913108190735e-31+sqrt(3.0).*q6d.*conj(q5).*4.879913108190735e-31-sqrt(3.0).*q6d.*conj(q6).*1.46397393245722e-30,q1d.*2.730577954033007e+5+q2d.*1.398366081578192e+5+q3d.*3.095751114833673e+5+q4d.*5.443043298181812e+4-q5d.*6.047936538546912e+4+q6d.*5.627568258912012e+4+sqrt(3.0).*q1d.*3.555581400000001e+4+sqrt(3.0).*q2d.*3.30182648e+4+sqrt(3.0).*q3d.*6.09614312e+4+sqrt(3.0).*q4d.*4.54242006e+4+sqrt(3.0).*q5d.*1.50919214e+4+sqrt(3.0).*q6d.*1.494348499999999e+4+q1d.*conj(q1).*6.588133886663567e-14+q1d.*conj(q2).*6.588133886663567e-14+q2d.*conj(q1).*3.294066943331783e-14+q1d.*conj(q3).*1.07592391394e+3+q2d.*conj(q2).*6.588133886663567e-14+q3d.*conj(q1).*6.588133886663567e-14+q1d.*conj(q4).*4.3246e+2+q2d.*conj(q3).*1.07592391394e+3+q3d.*conj(q2).*6.588133886663567e-14+q4d.*conj(q1).*1.324026886898161e-14-q1d.*conj(q5).*3.9798e+2+q2d.*conj(q4).*4.3246e+2+q3d.*conj(q3).*2.15184782788e+3+q4d.*conj(q2).*1.324026886898161e-14-q5d.*conj(q1).*1.218462332811659e-14+q1d.*conj(q6).*3.635000000000001e+2-q2d.*conj(q5).*3.9798e+2+q3d.*conj(q4).*8.6492e+2+q4d.*conj(q3).*4.3246e+2-q5d.*conj(q2).*1.218462332811659e-14+q6d.*conj(q1).*3.338693336175472e-14+q2d.*conj(q6).*3.635e+2-q3d.*conj(q5).*7.9596e+2+q4d.*conj(q4).*1.08115e+3-q5d.*conj(q3).*3.9798e+2+q6d.*conj(q2).*3.338693336175472e-14+q3d.*conj(q6).*7.27e+2+q4d.*conj(q5).*1.9899e+2+q5d.*conj(q4).*3.9798e+2+q6d.*conj(q3).*3.635e+2-q4d.*conj(q6).*1.8175e+2+q5d.*conj(q5).*5.9697e+2-q6d.*conj(q4).*3.635e+2-q5d.*conj(q6).*5.4525e+2-q6d.*conj(q5).*7.27e+2+q6d.*conj(q6).*9.0875e+2-sqrt(3.0).*q1d.*conj(q4).*4.3246e+2-sqrt(3.0).*q4d.*conj(q1).*2.1623e+2-sqrt(3.0).*q1d.*conj(q5).*3.9798e+2-sqrt(3.0).*q2d.*conj(q4).*2.1623e+2-sqrt(3.0).*q4d.*conj(q2).*2.1623e+2-sqrt(3.0).*q5d.*conj(q1).*1.9899e+2+sqrt(3.0).*q1d.*conj(q6).*3.635e+2-sqrt(3.0).*q2d.*conj(q5).*1.9899e+2+sqrt(3.0).*q3d.*conj(q4).*5.805686995235668e-31+sqrt(3.0).*q4d.*conj(q3).*2.902843497617834e-31-sqrt(3.0).*q5d.*conj(q2).*1.9899e+2+sqrt(3.0).*q6d.*conj(q1).*1.8175e+2+sqrt(3.0).*q2d.*conj(q6).*1.8175e+2+sqrt(3.0).*q3d.*conj(q5).*5.342800051713201e-31+sqrt(3.0).*q4d.*conj(q4).*4.354265246426751e-31+sqrt(3.0).*q5d.*conj(q3).*2.671400025856601e-31+sqrt(3.0).*q6d.*conj(q2).*1.8175e+2-sqrt(3.0).*q3d.*conj(q6).*8.903182229801258e-14+sqrt(3.0).*q4d.*conj(q5).*1.3357000129283e-31-sqrt(3.0).*q6d.*conj(q3).*4.451591114900629e-14-sqrt(3.0).*q4d.*conj(q6).*6.677386672350943e-14-sqrt(3.0).*q5d.*conj(q5).*1.3357000129283e-31-sqrt(3.0).*q6d.*conj(q4).*4.451591114900629e-14-sqrt(3.0).*q5d.*conj(q6).*2.225795557450314e-14+sqrt(3.0).*q6d.*conj(q5).*4.879913108190735e-31-sqrt(3.0).*q6d.*conj(q6).*2.225795557450315e-14,q1d.*1.398366081578192e+5-q2d.*2.328647425539134e+4+q3d.*1.323084182467521e+4-q4d.*5.126307600000002e+3-q5d.*5.671078800000006e+3+q6d.*6.215850000000002e+3+sqrt(3.0).*q1d.*3.30182648e+4+sqrt(3.0).*q2d.*3.555581400000001e+4+sqrt(3.0).*q3d.*6.09614312e+4+sqrt(3.0).*q4d.*4.54242006e+4+sqrt(3.0).*q5d.*1.50919214e+4+sqrt(3.0).*q6d.*1.4943485e+4+q1d.*conj(q1).*3.294066943331783e-14+q1d.*conj(q2).*6.588133886663567e-14+q1d.*conj(q3).*1.07592391394e+3+q2d.*conj(q2).*6.588133886663567e-14+q1d.*conj(q4).*4.3246e+2+q2d.*conj(q3).*1.07592391394e+3+q3d.*conj(q2).*6.588133886663567e-14-q1d.*conj(q5).*3.9798e+2+q2d.*conj(q4).*4.3246e+2+q3d.*conj(q3).*2.15184782788e+3+q4d.*conj(q2).*1.324026886898161e-14+q1d.*conj(q6).*3.635e+2-q2d.*conj(q5).*3.9798e+2+q3d.*conj(q4).*8.6492e+2+q4d.*conj(q3).*4.3246e+2-q5d.*conj(q2).*1.218462332811659e-14+q2d.*conj(q6).*3.635000000000001e+2-q3d.*conj(q5).*7.9596e+2+q4d.*conj(q4).*1.08115e+3-q5d.*conj(q3).*3.9798e+2+q6d.*conj(q2).*3.338693336175472e-14+q3d.*conj(q6).*7.27e+2+q4d.*conj(q5).*1.9899e+2+q5d.*conj(q4).*3.9798e+2+q6d.*conj(q3).*3.635e+2-q4d.*conj(q6).*1.8175e+2+q5d.*conj(q5).*5.9697e+2-q6d.*conj(q4).*3.635e+2-q5d.*conj(q6).*5.4525e+2-q6d.*conj(q5).*7.27e+2+q6d.*conj(q6).*9.0875e+2-sqrt(3.0).*q1d.*conj(q4).*2.1623e+2-sqrt(3.0).*q1d.*conj(q5).*1.9899e+2-sqrt(3.0).*q2d.*conj(q4).*4.3246e+2-sqrt(3.0).*q4d.*conj(q2).*2.1623e+2+sqrt(3.0).*q1d.*conj(q6).*1.8175e+2-sqrt(3.0).*q2d.*conj(q5).*3.9798e+2+sqrt(3.0).*q3d.*conj(q4).*5.805686995235668e-31+sqrt(3.0).*q4d.*conj(q3).*2.902843497617834e-31-sqrt(3.0).*q5d.*conj(q2).*1.9899e+2+sqrt(3.0).*q2d.*conj(q6).*3.635e+2+sqrt(3.0).*q3d.*conj(q5).*5.342800051713201e-31+sqrt(3.0).*q4d.*conj(q4).*4.354265246426751e-31+sqrt(3.0).*q5d.*conj(q3).*2.671400025856601e-31+sqrt(3.0).*q6d.*conj(q2).*1.8175e+2-sqrt(3.0).*q3d.*conj(q6).*8.903182229801258e-14+sqrt(3.0).*q4d.*conj(q5).*1.3357000129283e-31-sqrt(3.0).*q6d.*conj(q3).*4.451591114900629e-14-sqrt(3.0).*q4d.*conj(q6).*6.677386672350943e-14-sqrt(3.0).*q5d.*conj(q5).*1.3357000129283e-31-sqrt(3.0).*q6d.*conj(q4).*4.451591114900629e-14-sqrt(3.0).*q5d.*conj(q6).*2.225795557450314e-14+sqrt(3.0).*q6d.*conj(q5).*4.879913108190735e-31-sqrt(3.0).*q6d.*conj(q6).*2.225795557450315e-14,q1d.*3.095751114833673e+5+q2d.*1.323084182467521e+4+q3d.*1.984626273701281e+4-q4d.*3.8831376e+3-q5d.*3.780719200000004e+3+q6d.*7.459020000000004e+3+sqrt(3.0).*q1d.*6.09614312e+4+sqrt(3.0).*q2d.*6.09614312e+4+sqrt(3.0).*q3d.*9.14421468e+4+sqrt(3.0).*q4d.*6.06645584e+4+sqrt(3.0).*q5d.*3.01838428e+4+sqrt(3.0).*q6d.*2.988697e+4+q1d.*conj(q1).*6.588133886663567e-14+q1d.*conj(q2).*6.588133886663567e-14+q1d.*conj(q3).*2.15184782788e+3+q2d.*conj(q2).*6.588133886663567e-14+q1d.*conj(q4).*8.6492e+2+q2d.*conj(q3).*2.15184782788e+3-q1d.*conj(q5).*7.9596e+2+q2d.*conj(q4).*8.6492e+2+q3d.*conj(q3).*3.22777174182e+3+q1d.*conj(q6).*7.27e+2-q2d.*conj(q5).*7.9596e+2+q3d.*conj(q4).*1.29738e+3+q4d.*conj(q3).*4.3246e+2+q2d.*conj(q6).*7.27e+2-q3d.*conj(q5).*1.19394e+3+q4d.*conj(q4).*1.29738e+3-q5d.*conj(q3).*3.9798e+2+q3d.*conj(q6).*1.0905e+3-q4d.*conj(q5).*6.544090984559467e-15+q5d.*conj(q4).*3.9798e+2+q6d.*conj(q3).*3.635e+2+q4d.*conj(q6).*5.977127174449385e-15+q5d.*conj(q5).*3.9798e+2-q6d.*conj(q4).*3.635e+2-q5d.*conj(q6).*3.635e+2-q6d.*conj(q5).*7.27e+2+q6d.*conj(q6).*1.0905e+3+sqrt(3.0).*q1d.*conj(q4).*5.805686995235668e-31+sqrt(3.0).*q1d.*conj(q5).*5.342800051713201e-31+sqrt(3.0).*q2d.*conj(q4).*5.805686995235668e-31-sqrt(3.0).*q1d.*conj(q6).*8.903182229801258e-14+sqrt(3.0).*q2d.*conj(q5).*5.342800051713201e-31+sqrt(3.0).*q3d.*conj(q4).*8.708530492853502e-31+sqrt(3.0).*q4d.*conj(q3).*2.902843497617834e-31-sqrt(3.0).*q2d.*conj(q6).*8.903182229801258e-14+sqrt(3.0).*q3d.*conj(q5).*8.014200077569802e-31+sqrt(3.0).*q4d.*conj(q4).*5.805686995235668e-31+sqrt(3.0).*q5d.*conj(q3).*2.671400025856601e-31-sqrt(3.0).*q3d.*conj(q6).*1.335477334470189e-13+sqrt(3.0).*q4d.*conj(q5).*2.671400025856601e-31-sqrt(3.0).*q6d.*conj(q3).*4.451591114900629e-14-sqrt(3.0).*q4d.*conj(q6).*8.903182229801258e-14-sqrt(3.0).*q6d.*conj(q4).*4.451591114900629e-14-sqrt(3.0).*q5d.*conj(q6).*4.451591114900629e-14+sqrt(3.0).*q6d.*conj(q5).*4.879913108190735e-31-sqrt(3.0).*q6d.*conj(q6).*4.451591114900629e-14,q1d.*5.443043298181812e+4-q2d.*5.126307600000002e+3-q3d.*3.8831376e+3-q4d.*1.273895520000001e+4-q5d.*9.451798000000009e+3+q6d.*3.729509999999998e+3+sqrt(3.0).*q1d.*4.54242006e+4+sqrt(3.0).*q2d.*4.54242006e+4+sqrt(3.0).*q3d.*6.06645584e+4+sqrt(3.0).*q4d.*6.03676856e+4+sqrt(3.0).*q5d.*1.50919214e+4+sqrt(3.0).*q6d.*1.4943485e+4+q1d.*conj(q1).*1.324026886898161e-14+q1d.*conj(q2).*1.324026886898161e-14+q1d.*conj(q3).*4.3246e+2+q2d.*conj(q2).*1.324026886898161e-14+q1d.*conj(q4).*1.08115e+3+q2d.*conj(q3).*4.3246e+2+q1d.*conj(q5).*1.9899e+2+q2d.*conj(q4).*1.08115e+3+q3d.*conj(q3).*4.3246e+2-q1d.*conj(q6).*1.8175e+2+q2d.*conj(q5).*1.9899e+2+q3d.*conj(q4).*1.29738e+3+q4d.*conj(q3).*4.3246e+2-q2d.*conj(q6).*1.8175e+2-q3d.*conj(q5).*6.544090984559467e-15+q4d.*conj(q4).*1.72984e+3-q5d.*conj(q3).*1.9899e+2+q3d.*conj(q6).*5.977127174449385e-15+q4d.*conj(q5).*7.9596e+2+q5d.*conj(q4).*3.9798e+2+q6d.*conj(q3).*1.8175e+2-q4d.*conj(q6).*7.27e+2+q5d.*conj(q5).*9.9495e+2-q6d.*conj(q4).*3.635e+2-q5d.*conj(q6).*9.0875e+2-q6d.*conj(q5).*7.27e+2+q6d.*conj(q6).*5.4525e+2-sqrt(3.0).*q1d.*conj(q1).*2.1623e+2-sqrt(3.0).*q1d.*conj(q2).*2.1623e+2+sqrt(3.0).*q1d.*conj(q3).*2.902843497617834e-31-sqrt(3.0).*q2d.*conj(q2).*2.1623e+2+sqrt(3.0).*q1d.*conj(q4).*4.354265246426751e-31+sqrt(3.0).*q2d.*conj(q3).*2.902843497617834e-31+sqrt(3.0).*q1d.*conj(q5).*1.3357000129283e-31+sqrt(3.0).*q2d.*conj(q4).*4.354265246426751e-31+sqrt(3.0).*q3d.*conj(q3).*2.902843497617834e-31-sqrt(3.0).*q1d.*conj(q6).*6.677386672350943e-14+sqrt(3.0).*q2d.*conj(q5).*1.3357000129283e-31+sqrt(3.0).*q3d.*conj(q4).*5.805686995235668e-31+sqrt(3.0).*q4d.*conj(q3).*2.902843497617834e-31-sqrt(3.0).*q2d.*conj(q6).*6.677386672350943e-14+sqrt(3.0).*q3d.*conj(q5).*2.671400025856601e-31+sqrt(3.0).*q4d.*conj(q4).*5.805686995235668e-31+sqrt(3.0).*q5d.*conj(q3).*1.3357000129283e-31-sqrt(3.0).*q3d.*conj(q6).*8.903182229801258e-14-sqrt(3.0).*q6d.*conj(q3).*2.225795557450315e-14-sqrt(3.0).*q4d.*conj(q6).*8.903182229801258e-14-sqrt(3.0).*q5d.*conj(q5).*2.671400025856601e-31-sqrt(3.0).*q6d.*conj(q4).*4.451591114900629e-14-sqrt(3.0).*q5d.*conj(q6).*2.225795557450314e-14+sqrt(3.0).*q6d.*conj(q5).*4.879913108190735e-31-sqrt(3.0).*q6d.*conj(q6).*2.225795557450315e-14,q1d.*(-6.047936538546912e+4)-q2d.*5.671078800000006e+3-q3d.*3.780719200000004e+3-q4d.*9.451798000000009e+3-q5d.*1.512287680000001e+4+q6d.*2.486339999999996e+3+sqrt(3.0).*q1d.*1.50919214e+4+sqrt(3.0).*q2d.*1.50919214e+4+sqrt(3.0).*q3d.*3.01838428e+4+sqrt(3.0).*q4d.*1.50919214e+4-sqrt(3.0).*q5d.*3.308806364588508e-13+sqrt(3.0).*q6d.*8.190656604720473e-14-q1d.*conj(q1).*1.218462332811659e-14-q1d.*conj(q2).*1.218462332811659e-14-q1d.*conj(q3).*3.9798e+2-q2d.*conj(q2).*1.218462332811659e-14+q1d.*conj(q4).*3.9798e+2-q2d.*conj(q3).*3.9798e+2+q1d.*conj(q5).*5.9697e+2+q2d.*conj(q4).*3.9798e+2-q3d.*conj(q3).*3.9798e+2-q1d.*conj(q6).*5.4525e+2+q2d.*conj(q5).*5.9697e+2+q3d.*conj(q4).*3.9798e+2-q4d.*conj(q3).*1.9899e+2-q2d.*conj(q6).*5.4525e+2+q3d.*conj(q5).*3.9798e+2+q4d.*conj(q4).*3.9798e+2-q5d.*conj(q3).*3.9798e+2-q3d.*conj(q6).*3.635e+2+q4d.*conj(q5).*9.9495e+2+q5d.*conj(q4).*3.9798e+2+q6d.*conj(q3).*1.8175e+2-q4d.*conj(q6).*9.0875e+2+q5d.*conj(q5).*1.59192e+3-q6d.*conj(q4).*1.8175e+2-q5d.*conj(q6).*1.454e+3-q6d.*conj(q5).*7.27e+2+q6d.*conj(q6).*3.635e+2-sqrt(3.0).*q1d.*conj(q1).*1.9899e+2-sqrt(3.0).*q1d.*conj(q2).*1.9899e+2+sqrt(3.0).*q1d.*conj(q3).*2.671400025856601e-31-sqrt(3.0).*q2d.*conj(q2).*1.9899e+2+sqrt(3.0).*q2d.*conj(q3).*2.671400025856601e-31-sqrt(3.0).*q1d.*conj(q5).*1.3357000129283e-31+sqrt(3.0).*q3d.*conj(q3).*2.671400025856601e-31-sqrt(3.0).*q1d.*conj(q6).*2.225795557450314e-14-sqrt(3.0).*q2d.*conj(q5).*1.3357000129283e-31+sqrt(3.0).*q4d.*conj(q3).*1.3357000129283e-31-sqrt(3.0).*q2d.*conj(q6).*2.225795557450314e-14+sqrt(3.0).*q5d.*conj(q3).*2.671400025856601e-31-sqrt(3.0).*q3d.*conj(q6).*4.451591114900629e-14-sqrt(3.0).*q4d.*conj(q5).*2.671400025856601e-31-sqrt(3.0).*q6d.*conj(q3).*2.225795557450315e-14-sqrt(3.0).*q4d.*conj(q6).*2.225795557450314e-14-sqrt(3.0).*q5d.*conj(q5).*5.342800051713201e-31-sqrt(3.0).*q6d.*conj(q4).*2.225795557450314e-14+sqrt(3.0).*q5d.*conj(q6).*9.75982621638147e-31+sqrt(3.0).*q6d.*conj(q5).*4.879913108190735e-31-sqrt(3.0).*q6d.*conj(q6).*4.879913108190735e-31,q1d.*5.627568258912012e+4+q2d.*6.215850000000002e+3+q3d.*7.459020000000004e+3+q4d.*3.729509999999998e+3+q5d.*2.486339999999996e+3+q6d.*9.94536e+3+sqrt(3.0).*q1d.*1.494348499999999e+4+sqrt(3.0).*q2d.*1.4943485e+4+sqrt(3.0).*q3d.*2.988697e+4+sqrt(3.0).*q4d.*1.4943485e+4+sqrt(3.0).*q5d.*8.190656604720473e-14+sqrt(3.0).*q6d.*3.276262641888189e-13+q1d.*conj(q1).*3.338693336175472e-14+q1d.*conj(q2).*3.338693336175472e-14+q1d.*conj(q3).*3.635e+2+q2d.*conj(q2).*3.338693336175472e-14-q1d.*conj(q4).*3.635e+2+q2d.*conj(q3).*3.635e+2-q1d.*conj(q5).*7.27e+2-q2d.*conj(q4).*3.635e+2+q3d.*conj(q3).*3.635e+2+q1d.*conj(q6).*9.0875e+2-q2d.*conj(q5).*7.27e+2-q3d.*conj(q4).*3.635e+2+q4d.*conj(q3).*1.8175e+2+q2d.*conj(q6).*9.0875e+2-q3d.*conj(q5).*7.27e+2-q4d.*conj(q4).*3.635e+2+q5d.*conj(q3).*1.8175e+2+q3d.*conj(q6).*1.0905e+3-q4d.*conj(q5).*7.27e+2-q5d.*conj(q4).*1.8175e+2+q6d.*conj(q3).*3.635e+2+q4d.*conj(q6).*5.4525e+2-q5d.*conj(q5).*7.27e+2-q6d.*conj(q4).*3.635e+2+q5d.*conj(q6).*3.635e+2-q6d.*conj(q5).*7.27e+2+q6d.*conj(q6).*1.454e+3+sqrt(3.0).*q1d.*conj(q1).*1.8175e+2+sqrt(3.0).*q1d.*conj(q2).*1.8175e+2-sqrt(3.0).*q1d.*conj(q3).*4.451591114900629e-14+sqrt(3.0).*q2d.*conj(q2).*1.8175e+2-sqrt(3.0).*q1d.*conj(q4).*4.451591114900629e-14-sqrt(3.0).*q2d.*conj(q3).*4.451591114900629e-14+sqrt(3.0).*q1d.*conj(q5).*4.879913108190735e-31-sqrt(3.0).*q2d.*conj(q4).*4.451591114900629e-14-sqrt(3.0).*q3d.*conj(q3).*4.451591114900629e-14-sqrt(3.0).*q1d.*conj(q6).*2.225795557450315e-14+sqrt(3.0).*q2d.*conj(q5).*4.879913108190735e-31-sqrt(3.0).*q3d.*conj(q4).*4.451591114900629e-14-sqrt(3.0).*q4d.*conj(q3).*2.225795557450315e-14-sqrt(3.0).*q2d.*conj(q6).*2.225795557450315e-14+sqrt(3.0).*q3d.*conj(q5).*4.879913108190735e-31-sqrt(3.0).*q4d.*conj(q4).*4.451591114900629e-14-sqrt(3.0).*q5d.*conj(q3).*2.225795557450315e-14-sqrt(3.0).*q3d.*conj(q6).*4.451591114900629e-14+sqrt(3.0).*q4d.*conj(q5).*4.879913108190735e-31-sqrt(3.0).*q5d.*conj(q4).*2.225795557450314e-14-sqrt(3.0).*q6d.*conj(q3).*4.451591114900629e-14-sqrt(3.0).*q4d.*conj(q6).*2.225795557450315e-14+sqrt(3.0).*q5d.*conj(q5).*4.879913108190735e-31-sqrt(3.0).*q6d.*conj(q4).*4.451591114900629e-14-sqrt(3.0).*q5d.*conj(q6).*4.879913108190735e-31+sqrt(3.0).*q6d.*conj(q5).*4.879913108190735e-31-sqrt(3.0).*q6d.*conj(q6).*1.46397393245722e-30,q1d.*8.285703356363623e+4+q2d.*3.824377798181812e+4+q3d.*5.443043298181812e+4+q4d.*1.063745259636362e+5-q5d.*6.426008458546913e+4+q6d.*5.378934258912012e+4+sqrt(3.0).*q1d.*3.525894120000001e+4+sqrt(3.0).*q2d.*3.272139200000001e+4+sqrt(3.0).*q3d.*4.54242006e+4+sqrt(3.0).*q4d.*6.036768560000001e+4+sqrt(3.0).*q5d.*1.50919214e+4+sqrt(3.0).*q6d.*1.494348499999999e+4+q1d.*conj(q1).*2.648053773796322e-14+q1d.*conj(q2).*2.648053773796322e-14+q2d.*conj(q1).*1.324026886898161e-14+q1d.*conj(q3).*4.3246e+2+q2d.*conj(q2).*2.648053773796322e-14+q3d.*conj(q1).*1.324026886898161e-14+q1d.*conj(q4).*8.6492e+2+q2d.*conj(q3).*4.3246e+2+q3d.*conj(q2).*1.324026886898161e-14+q4d.*conj(q1).*2.648053773796322e-14+q1d.*conj(q5).*3.9798e+2+q2d.*conj(q4).*8.6492e+2+q3d.*conj(q3).*4.3246e+2+q4d.*conj(q2).*2.648053773796322e-14-q5d.*conj(q1).*1.218462332811659e-14-q1d.*conj(q6).*3.634999999999999e+2+q2d.*conj(q5).*3.9798e+2+q3d.*conj(q4).*1.08115e+3+q4d.*conj(q3).*4.3246e+2-q5d.*conj(q2).*1.218462332811659e-14+q6d.*conj(q1).*3.338693336175472e-14-q2d.*conj(q6).*3.635e+2+q3d.*conj(q5).*1.9899e+2+q4d.*conj(q4).*1.72984e+3-q5d.*conj(q3).*1.9899e+2+q6d.*conj(q2).*3.338693336175472e-14-q3d.*conj(q6).*1.8175e+2+q4d.*conj(q5).*7.9596e+2+q5d.*conj(q4).*3.9798e+2+q6d.*conj(q3).*1.8175e+2-q4d.*conj(q6).*7.27e+2+q5d.*conj(q5).*9.9495e+2-q6d.*conj(q4).*3.635e+2-q5d.*conj(q6).*9.0875e+2-q6d.*conj(q5).*7.27e+2+q6d.*conj(q6).*5.4525e+2-sqrt(3.0).*q1d.*conj(q1).*4.3246e+2-sqrt(3.0).*q1d.*conj(q2).*4.3246e+2-sqrt(3.0).*q2d.*conj(q1).*2.1623e+2+sqrt(3.0).*q1d.*conj(q3).*2.902843497617834e-31-sqrt(3.0).*q2d.*conj(q2).*4.3246e+2-sqrt(3.0).*q3d.*conj(q1).*2.1623e+2-sqrt(3.0).*q1d.*conj(q4).*4.3246e+2+sqrt(3.0).*q2d.*conj(q3).*2.902843497617834e-31-sqrt(3.0).*q3d.*conj(q2).*2.1623e+2-sqrt(3.0).*q4d.*conj(q1).*4.3246e+2-sqrt(3.0).*q1d.*conj(q5).*3.9798e+2-sqrt(3.0).*q2d.*conj(q4).*2.1623e+2+sqrt(3.0).*q3d.*conj(q3).*2.902843497617834e-31-sqrt(3.0).*q4d.*conj(q2).*4.3246e+2-sqrt(3.0).*q5d.*conj(q1).*1.9899e+2+sqrt(3.0).*q1d.*conj(q6).*3.635e+2-sqrt(3.0).*q2d.*conj(q5).*1.9899e+2+sqrt(3.0).*q3d.*conj(q4).*4.354265246426751e-31+sqrt(3.0).*q4d.*conj(q3).*2.902843497617834e-31-sqrt(3.0).*q5d.*conj(q2).*1.9899e+2+sqrt(3.0).*q6d.*conj(q1).*1.8175e+2+sqrt(3.0).*q2d.*conj(q6).*1.8175e+2+sqrt(3.0).*q3d.*conj(q5).*1.3357000129283e-31+sqrt(3.0).*q4d.*conj(q4).*5.805686995235668e-31+sqrt(3.0).*q5d.*conj(q3).*1.3357000129283e-31+sqrt(3.0).*q6d.*conj(q2).*1.8175e+2-sqrt(3.0).*q3d.*conj(q6).*6.677386672350943e-14-sqrt(3.0).*q6d.*conj(q3).*2.225795557450315e-14-sqrt(3.0).*q4d.*conj(q6).*8.903182229801258e-14-sqrt(3.0).*q5d.*conj(q5).*2.671400025856601e-31-sqrt(3.0).*q6d.*conj(q4).*4.451591114900629e-14-sqrt(3.0).*q5d.*conj(q6).*2.225795557450314e-14+sqrt(3.0).*q6d.*conj(q5).*4.879913108190735e-31-sqrt(3.0).*q6d.*conj(q6).*2.225795557450315e-14,q1d.*3.824377798181812e+4-q2d.*3.62564476e+4-q3d.*5.126307600000002e+3-q4d.*1.273895520000001e+4-q5d.*9.451798000000009e+3+q6d.*3.729509999999998e+3+sqrt(3.0).*q1d.*3.272139200000001e+4+sqrt(3.0).*q2d.*3.525894120000001e+4+sqrt(3.0).*q3d.*4.54242006e+4+sqrt(3.0).*q4d.*6.03676856e+4+sqrt(3.0).*q5d.*1.50919214e+4+sqrt(3.0).*q6d.*1.4943485e+4+q1d.*conj(q1).*1.324026886898161e-14+q1d.*conj(q2).*2.648053773796322e-14+q1d.*conj(q3).*4.3246e+2+q2d.*conj(q2).*2.648053773796322e-14+q1d.*conj(q4).*8.6492e+2+q2d.*conj(q3).*4.3246e+2+q3d.*conj(q2).*1.324026886898161e-14+q1d.*conj(q5).*3.9798e+2+q2d.*conj(q4).*8.6492e+2+q3d.*conj(q3).*4.3246e+2+q4d.*conj(q2).*2.648053773796322e-14-q1d.*conj(q6).*3.635e+2+q2d.*conj(q5).*3.9798e+2+q3d.*conj(q4).*1.08115e+3+q4d.*conj(q3).*4.3246e+2-q5d.*conj(q2).*1.218462332811659e-14-q2d.*conj(q6).*3.634999999999999e+2+q3d.*conj(q5).*1.9899e+2+q4d.*conj(q4).*1.72984e+3-q5d.*conj(q3).*1.9899e+2+q6d.*conj(q2).*3.338693336175472e-14-q3d.*conj(q6).*1.8175e+2+q4d.*conj(q5).*7.9596e+2+q5d.*conj(q4).*3.9798e+2+q6d.*conj(q3).*1.8175e+2-q4d.*conj(q6).*7.27e+2+q5d.*conj(q5).*9.9495e+2-q6d.*conj(q4).*3.635e+2-q5d.*conj(q6).*9.0875e+2-q6d.*conj(q5).*7.27e+2+q6d.*conj(q6).*5.4525e+2-sqrt(3.0).*q1d.*conj(q1).*2.1623e+2-sqrt(3.0).*q1d.*conj(q2).*4.3246e+2+sqrt(3.0).*q1d.*conj(q3).*2.902843497617834e-31-sqrt(3.0).*q2d.*conj(q2).*4.3246e+2-sqrt(3.0).*q1d.*conj(q4).*2.1623e+2+sqrt(3.0).*q2d.*conj(q3).*2.902843497617834e-31-sqrt(3.0).*q3d.*conj(q2).*2.1623e+2-sqrt(3.0).*q1d.*conj(q5).*1.9899e+2-sqrt(3.0).*q2d.*conj(q4).*4.3246e+2+sqrt(3.0).*q3d.*conj(q3).*2.902843497617834e-31-sqrt(3.0).*q4d.*conj(q2).*4.3246e+2+sqrt(3.0).*q1d.*conj(q6).*1.8175e+2-sqrt(3.0).*q2d.*conj(q5).*3.9798e+2+sqrt(3.0).*q3d.*conj(q4).*4.354265246426751e-31+sqrt(3.0).*q4d.*conj(q3).*2.902843497617834e-31-sqrt(3.0).*q5d.*conj(q2).*1.9899e+2+sqrt(3.0).*q2d.*conj(q6).*3.635e+2+sqrt(3.0).*q3d.*conj(q5).*1.3357000129283e-31+sqrt(3.0).*q4d.*conj(q4).*5.805686995235668e-31+sqrt(3.0).*q5d.*conj(q3).*1.3357000129283e-31+sqrt(3.0).*q6d.*conj(q2).*1.8175e+2-sqrt(3.0).*q3d.*conj(q6).*6.677386672350943e-14-sqrt(3.0).*q6d.*conj(q3).*2.225795557450315e-14-sqrt(3.0).*q4d.*conj(q6).*8.903182229801258e-14-sqrt(3.0).*q5d.*conj(q5).*2.671400025856601e-31-sqrt(3.0).*q6d.*conj(q4).*4.451591114900629e-14-sqrt(3.0).*q5d.*conj(q6).*2.225795557450314e-14+sqrt(3.0).*q6d.*conj(q5).*4.879913108190735e-31-sqrt(3.0).*q6d.*conj(q6).*2.225795557450315e-14,q1d.*5.443043298181812e+4-q2d.*5.126307600000002e+3-q3d.*3.8831376e+3-q4d.*1.273895520000001e+4-q5d.*9.451798000000009e+3+q6d.*3.729509999999998e+3+sqrt(3.0).*q1d.*4.54242006e+4+sqrt(3.0).*q2d.*4.54242006e+4+sqrt(3.0).*q3d.*6.06645584e+4+sqrt(3.0).*q4d.*6.03676856e+4+sqrt(3.0).*q5d.*1.50919214e+4+sqrt(3.0).*q6d.*1.4943485e+4+q1d.*conj(q1).*1.324026886898161e-14+q1d.*conj(q2).*1.324026886898161e-14+q1d.*conj(q3).*4.3246e+2+q2d.*conj(q2).*1.324026886898161e-14+q1d.*conj(q4).*1.08115e+3+q2d.*conj(q3).*4.3246e+2+q1d.*conj(q5).*1.9899e+2+q2d.*conj(q4).*1.08115e+3+q3d.*conj(q3).*4.3246e+2-q1d.*conj(q6).*1.8175e+2+q2d.*conj(q5).*1.9899e+2+q3d.*conj(q4).*1.29738e+3+q4d.*conj(q3).*4.3246e+2-q2d.*conj(q6).*1.8175e+2-q3d.*conj(q5).*6.544090984559467e-15+q4d.*conj(q4).*1.72984e+3-q5d.*conj(q3).*1.9899e+2+q3d.*conj(q6).*5.977127174449385e-15+q4d.*conj(q5).*7.9596e+2+q5d.*conj(q4).*3.9798e+2+q6d.*conj(q3).*1.8175e+2-q4d.*conj(q6).*7.27e+2+q5d.*conj(q5).*9.9495e+2-q6d.*conj(q4).*3.635e+2-q5d.*conj(q6).*9.0875e+2-q6d.*conj(q5).*7.27e+2+q6d.*conj(q6).*5.4525e+2-sqrt(3.0).*q1d.*conj(q1).*2.1623e+2-sqrt(3.0).*q1d.*conj(q2).*2.1623e+2+sqrt(3.0).*q1d.*conj(q3).*2.902843497617834e-31-sqrt(3.0).*q2d.*conj(q2).*2.1623e+2+sqrt(3.0).*q1d.*conj(q4).*4.354265246426751e-31+sqrt(3.0).*q2d.*conj(q3).*2.902843497617834e-31+sqrt(3.0).*q1d.*conj(q5).*1.3357000129283e-31+sqrt(3.0).*q2d.*conj(q4).*4.354265246426751e-31+sqrt(3.0).*q3d.*conj(q3).*2.902843497617834e-31-sqrt(3.0).*q1d.*conj(q6).*6.677386672350943e-14+sqrt(3.0).*q2d.*conj(q5).*1.3357000129283e-31+sqrt(3.0).*q3d.*conj(q4).*5.805686995235668e-31+sqrt(3.0).*q4d.*conj(q3).*2.902843497617834e-31-sqrt(3.0).*q2d.*conj(q6).*6.677386672350943e-14+sqrt(3.0).*q3d.*conj(q5).*2.671400025856601e-31+sqrt(3.0).*q4d.*conj(q4).*5.805686995235668e-31+sqrt(3.0).*q5d.*conj(q3).*1.3357000129283e-31-sqrt(3.0).*q3d.*conj(q6).*8.903182229801258e-14-sqrt(3.0).*q6d.*conj(q3).*2.225795557450315e-14-sqrt(3.0).*q4d.*conj(q6).*8.903182229801258e-14-sqrt(3.0).*q5d.*conj(q5).*2.671400025856601e-31-sqrt(3.0).*q6d.*conj(q4).*4.451591114900629e-14-sqrt(3.0).*q5d.*conj(q6).*2.225795557450314e-14+sqrt(3.0).*q6d.*conj(q5).*4.879913108190735e-31-sqrt(3.0).*q6d.*conj(q6).*2.225795557450315e-14,q1d.*1.063745259636362e+5-q2d.*1.273895520000001e+4-q3d.*1.273895520000001e+4-q4d.*1.910843280000001e+4-q5d.*1.134215760000001e+4+q6d.*2.486339999999996e+3+sqrt(3.0).*q1d.*6.036768560000001e+4+sqrt(3.0).*q2d.*6.03676856e+4+sqrt(3.0).*q3d.*6.03676856e+4+sqrt(3.0).*q4d.*9.05515284e+4+sqrt(3.0).*q5d.*3.01838428e+4+sqrt(3.0).*q6d.*2.988697e+4+q1d.*conj(q1).*2.648053773796322e-14+q1d.*conj(q2).*2.648053773796322e-14+q1d.*conj(q3).*4.3246e+2+q2d.*conj(q2).*2.648053773796322e-14+q1d.*conj(q4).*1.72984e+3+q2d.*conj(q3).*4.3246e+2+q1d.*conj(q5).*7.9596e+2+q2d.*conj(q4).*1.72984e+3+q3d.*conj(q3).*4.3246e+2-q1d.*conj(q6).*7.27e+2+q2d.*conj(q5).*7.9596e+2+q3d.*conj(q4).*1.72984e+3-q2d.*conj(q6).*7.27e+2+q3d.*conj(q5).*7.9596e+2+q4d.*conj(q4).*2.59476e+3-q3d.*conj(q6).*7.27e+2+q4d.*conj(q5).*1.19394e+3+q5d.*conj(q4).*3.9798e+2-q4d.*conj(q6).*1.0905e+3+q5d.*conj(q5).*1.19394e+3-q6d.*conj(q4).*3.635e+2-q5d.*conj(q6).*1.0905e+3-q6d.*conj(q5).*7.27e+2+q6d.*conj(q6).*3.635e+2-sqrt(3.0).*q1d.*conj(q1).*4.3246e+2-sqrt(3.0).*q1d.*conj(q2).*4.3246e+2+sqrt(3.0).*q1d.*conj(q3).*2.902843497617834e-31-sqrt(3.0).*q2d.*conj(q2).*4.3246e+2+sqrt(3.0).*q1d.*conj(q4).*5.805686995235668e-31+sqrt(3.0).*q2d.*conj(q3).*2.902843497617834e-31+sqrt(3.0).*q2d.*conj(q4).*5.805686995235668e-31+sqrt(3.0).*q3d.*conj(q3).*2.902843497617834e-31-sqrt(3.0).*q1d.*conj(q6).*8.903182229801258e-14+sqrt(3.0).*q3d.*conj(q4).*5.805686995235668e-31-sqrt(3.0).*q2d.*conj(q6).*8.903182229801258e-14+sqrt(3.0).*q4d.*conj(q4).*8.708530492853502e-31-sqrt(3.0).*q3d.*conj(q6).*8.903182229801258e-14-sqrt(3.0).*q4d.*conj(q6).*1.335477334470189e-13-sqrt(3.0).*q5d.*conj(q5).*2.671400025856601e-31-sqrt(3.0).*q6d.*conj(q4).*4.451591114900629e-14-sqrt(3.0).*q5d.*conj(q6).*4.451591114900629e-14+sqrt(3.0).*q6d.*conj(q5).*4.879913108190735e-31-sqrt(3.0).*q6d.*conj(q6).*4.451591114900629e-14,q1d.*(-6.426008458546913e+4)-q2d.*9.451798000000009e+3-q3d.*9.451798000000009e+3-q4d.*1.134215760000001e+4-q5d.*1.512287680000001e+4+q6d.*2.486339999999996e+3+sqrt(3.0).*q1d.*1.50919214e+4+sqrt(3.0).*q2d.*1.50919214e+4+sqrt(3.0).*q3d.*1.50919214e+4+sqrt(3.0).*q4d.*3.01838428e+4-sqrt(3.0).*q5d.*3.308806364588508e-13+sqrt(3.0).*q6d.*8.190656604720473e-14-q1d.*conj(q1).*1.218462332811659e-14-q1d.*conj(q2).*1.218462332811659e-14-q1d.*conj(q3).*1.9899e+2-q2d.*conj(q2).*1.218462332811659e-14+q1d.*conj(q4).*3.9798e+2-q2d.*conj(q3).*1.9899e+2+q1d.*conj(q5).*9.9495e+2+q2d.*conj(q4).*3.9798e+2-q3d.*conj(q3).*1.9899e+2-q1d.*conj(q6).*9.0875e+2+q2d.*conj(q5).*9.9495e+2+q3d.*conj(q4).*3.9798e+2-q2d.*conj(q6).*9.0875e+2+q3d.*conj(q5).*9.9495e+2+q4d.*conj(q4).*3.9798e+2-q3d.*conj(q6).*9.0875e+2+q4d.*conj(q5).*1.19394e+3+q5d.*conj(q4).*3.9798e+2-q4d.*conj(q6).*1.0905e+3+q5d.*conj(q5).*1.59192e+3-q6d.*conj(q4).*1.8175e+2-q5d.*conj(q6).*1.454e+3-q6d.*conj(q5).*7.27e+2+q6d.*conj(q6).*3.635e+2-sqrt(3.0).*q1d.*conj(q1).*1.9899e+2-sqrt(3.0).*q1d.*conj(q2).*1.9899e+2+sqrt(3.0).*q1d.*conj(q3).*1.3357000129283e-31-sqrt(3.0).*q2d.*conj(q2).*1.9899e+2+sqrt(3.0).*q2d.*conj(q3).*1.3357000129283e-31-sqrt(3.0).*q1d.*conj(q5).*2.671400025856601e-31+sqrt(3.0).*q3d.*conj(q3).*1.3357000129283e-31-sqrt(3.0).*q1d.*conj(q6).*2.225795557450314e-14-sqrt(3.0).*q2d.*conj(q5).*2.671400025856601e-31-sqrt(3.0).*q2d.*conj(q6).*2.225795557450314e-14-sqrt(3.0).*q3d.*conj(q5).*2.671400025856601e-31-sqrt(3.0).*q3d.*conj(q6).*2.225795557450314e-14-sqrt(3.0).*q4d.*conj(q5).*2.671400025856601e-31-sqrt(3.0).*q4d.*conj(q6).*4.451591114900629e-14-sqrt(3.0).*q5d.*conj(q5).*5.342800051713201e-31-sqrt(3.0).*q6d.*conj(q4).*2.225795557450314e-14+sqrt(3.0).*q5d.*conj(q6).*9.75982621638147e-31+sqrt(3.0).*q6d.*conj(q5).*4.879913108190735e-31-sqrt(3.0).*q6d.*conj(q6).*4.879913108190735e-31,q1d.*5.378934258912012e+4+q2d.*3.729509999999998e+3+q3d.*3.729509999999998e+3+q4d.*2.486339999999996e+3+q5d.*2.486339999999996e+3+q6d.*9.94536e+3+sqrt(3.0).*q1d.*1.494348499999999e+4+sqrt(3.0).*q2d.*1.4943485e+4+sqrt(3.0).*q3d.*1.4943485e+4+sqrt(3.0).*q4d.*2.988697e+4+sqrt(3.0).*q5d.*8.190656604720473e-14+sqrt(3.0).*q6d.*3.276262641888189e-13+q1d.*conj(q1).*3.338693336175472e-14+q1d.*conj(q2).*3.338693336175472e-14+q1d.*conj(q3).*1.8175e+2+q2d.*conj(q2).*3.338693336175472e-14-q1d.*conj(q4).*3.635e+2+q2d.*conj(q3).*1.8175e+2-q1d.*conj(q5).*7.27e+2-q2d.*conj(q4).*3.635e+2+q3d.*conj(q3).*1.8175e+2+q1d.*conj(q6).*5.4525e+2-q2d.*conj(q5).*7.27e+2-q3d.*conj(q4).*3.635e+2+q2d.*conj(q6).*5.4525e+2-q3d.*conj(q5).*7.27e+2-q4d.*conj(q4).*3.635e+2+q3d.*conj(q6).*5.4525e+2-q4d.*conj(q5).*7.27e+2-q5d.*conj(q4).*1.8175e+2+q4d.*conj(q6).*3.635e+2-q5d.*conj(q5).*7.27e+2-q6d.*conj(q4).*3.635e+2+q5d.*conj(q6).*3.635e+2-q6d.*conj(q5).*7.27e+2+q6d.*conj(q6).*1.454e+3+sqrt(3.0).*q1d.*conj(q1).*1.8175e+2+sqrt(3.0).*q1d.*conj(q2).*1.8175e+2-sqrt(3.0).*q1d.*conj(q3).*2.225795557450315e-14+sqrt(3.0).*q2d.*conj(q2).*1.8175e+2-sqrt(3.0).*q1d.*conj(q4).*4.451591114900629e-14-sqrt(3.0).*q2d.*conj(q3).*2.225795557450315e-14+sqrt(3.0).*q1d.*conj(q5).*4.879913108190735e-31-sqrt(3.0).*q2d.*conj(q4).*4.451591114900629e-14-sqrt(3.0).*q3d.*conj(q3).*2.225795557450315e-14-sqrt(3.0).*q1d.*conj(q6).*2.225795557450315e-14+sqrt(3.0).*q2d.*conj(q5).*4.879913108190735e-31-sqrt(3.0).*q3d.*conj(q4).*4.451591114900629e-14-sqrt(3.0).*q2d.*conj(q6).*2.225795557450315e-14+sqrt(3.0).*q3d.*conj(q5).*4.879913108190735e-31-sqrt(3.0).*q4d.*conj(q4).*4.451591114900629e-14-sqrt(3.0).*q3d.*conj(q6).*2.225795557450315e-14+sqrt(3.0).*q4d.*conj(q5).*4.879913108190735e-31-sqrt(3.0).*q5d.*conj(q4).*2.225795557450314e-14-sqrt(3.0).*q4d.*conj(q6).*4.451591114900629e-14+sqrt(3.0).*q5d.*conj(q5).*4.879913108190735e-31-sqrt(3.0).*q6d.*conj(q4).*4.451591114900629e-14-sqrt(3.0).*q5d.*conj(q6).*4.879913108190735e-31+sqrt(3.0).*q6d.*conj(q5).*4.879913108190735e-31-sqrt(3.0).*q6d.*conj(q6).*1.46397393245722e-30,q1d.*(-1.473618543709382e+5)-q2d.*7.746164638546913e+4-q3d.*6.047936538546912e+4-q4d.*6.426008458546913e+4-q5d.*1.247394499709383e+5+q6d.*5.254617258912011e+4+sqrt(3.0).*q1d.*3.780719200000012e+3+sqrt(3.0).*q2d.*1.890359600000006e+3+sqrt(3.0).*q3d.*1.50919214e+4+sqrt(3.0).*q4d.*1.50919214e+4+sqrt(3.0).*q5d.*6.381198636905707e-12-sqrt(3.0).*q6d.*9.113935495870542e-12-q1d.*conj(q1).*2.436924665623318e-14-q1d.*conj(q2).*2.436924665623318e-14-q2d.*conj(q1).*1.218462332811659e-14-q1d.*conj(q3).*3.9798e+2-q2d.*conj(q2).*2.436924665623318e-14-q3d.*conj(q1).*1.218462332811659e-14+q1d.*conj(q4).*3.9798e+2-q2d.*conj(q3).*3.9798e+2-q3d.*conj(q2).*1.218462332811659e-14-q4d.*conj(q1).*1.218462332811659e-14+q1d.*conj(q5).*7.9596e+2+q2d.*conj(q4).*3.9798e+2-q3d.*conj(q3).*3.9798e+2-q4d.*conj(q2).*1.218462332811659e-14-q5d.*conj(q1).*2.436924665623318e-14-q1d.*conj(q6).*7.269999999999999e+2+q2d.*conj(q5).*7.9596e+2+q3d.*conj(q4).*3.9798e+2-q4d.*conj(q3).*1.9899e+2-q5d.*conj(q2).*2.436924665623318e-14+q6d.*conj(q1).*3.338693336175472e-14-q2d.*conj(q6).*7.27e+2+q3d.*conj(q5).*5.9697e+2+q4d.*conj(q4).*3.9798e+2-q5d.*conj(q3).*3.9798e+2+q6d.*conj(q2).*3.338693336175472e-14-q3d.*conj(q6).*5.4525e+2+q4d.*conj(q5).*9.9495e+2+q5d.*conj(q4).*3.9798e+2+q6d.*conj(q3).*1.8175e+2-q4d.*conj(q6).*9.0875e+2+q5d.*conj(q5).*1.59192e+3-q6d.*conj(q4).*1.8175e+2-q5d.*conj(q6).*1.454e+3-q6d.*conj(q5).*7.27e+2+q6d.*conj(q6).*3.635e+2-sqrt(3.0).*q1d.*conj(q1).*3.9798e+2-sqrt(3.0).*q1d.*conj(q2).*3.9798e+2-sqrt(3.0).*q2d.*conj(q1).*1.9899e+2+sqrt(3.0).*q1d.*conj(q3).*2.671400025856601e-31-sqrt(3.0).*q2d.*conj(q2).*3.9798e+2-sqrt(3.0).*q3d.*conj(q1).*1.9899e+2+sqrt(3.0).*q2d.*conj(q3).*2.671400025856601e-31-sqrt(3.0).*q3d.*conj(q2).*1.9899e+2-sqrt(3.0).*q4d.*conj(q1).*1.9899e+2-sqrt(3.0).*q1d.*conj(q5).*3.9798e+2+sqrt(3.0).*q3d.*conj(q3).*2.671400025856601e-31-sqrt(3.0).*q4d.*conj(q2).*1.9899e+2-sqrt(3.0).*q5d.*conj(q1).*3.9798e+2+sqrt(3.0).*q1d.*conj(q6).*3.635e+2-sqrt(3.0).*q2d.*conj(q5).*1.9899e+2+sqrt(3.0).*q4d.*conj(q3).*1.3357000129283e-31-sqrt(3.0).*q5d.*conj(q2).*3.9798e+2+sqrt(3.0).*q6d.*conj(q1).*1.8175e+2+sqrt(3.0).*q2d.*conj(q6).*1.8175e+2-sqrt(3.0).*q3d.*conj(q5).*1.3357000129283e-31+sqrt(3.0).*q5d.*conj(q3).*2.671400025856601e-31+sqrt(3.0).*q6d.*conj(q2).*1.8175e+2-sqrt(3.0).*q3d.*conj(q6).*2.225795557450314e-14-sqrt(3.0).*q4d.*conj(q5).*2.671400025856601e-31-sqrt(3.0).*q6d.*conj(q3).*2.225795557450315e-14-sqrt(3.0).*q4d.*conj(q6).*2.225795557450314e-14-sqrt(3.0).*q5d.*conj(q5).*5.342800051713201e-31-sqrt(3.0).*q6d.*conj(q4).*2.225795557450314e-14+sqrt(3.0).*q5d.*conj(q6).*9.75982621638147e-31+sqrt(3.0).*q6d.*conj(q5).*4.879913108190735e-31-sqrt(3.0).*q6d.*conj(q6).*4.879913108190735e-31,q1d.*(-7.746164638546913e+4)-q2d.*3.774528120000001e+4-q3d.*5.671078800000006e+3-q4d.*9.451798000000009e+3-q5d.*1.512287680000001e+4+q6d.*2.486339999999996e+3+sqrt(3.0).*q1d.*1.890359600000006e+3+sqrt(3.0).*q2d.*3.780719200000005e+3+sqrt(3.0).*q3d.*1.50919214e+4+sqrt(3.0).*q4d.*1.50919214e+4-sqrt(3.0).*q5d.*3.308806364588508e-13+sqrt(3.0).*q6d.*8.190656604720473e-14-q1d.*conj(q1).*1.218462332811659e-14-q1d.*conj(q2).*2.436924665623318e-14-q1d.*conj(q3).*3.9798e+2-q2d.*conj(q2).*2.436924665623318e-14+q1d.*conj(q4).*3.9798e+2-q2d.*conj(q3).*3.9798e+2-q3d.*conj(q2).*1.218462332811659e-14+q1d.*conj(q5).*7.9596e+2+q2d.*conj(q4).*3.9798e+2-q3d.*conj(q3).*3.9798e+2-q4d.*conj(q2).*1.218462332811659e-14-q1d.*conj(q6).*7.27e+2+q2d.*conj(q5).*7.9596e+2+q3d.*conj(q4).*3.9798e+2-q4d.*conj(q3).*1.9899e+2-q5d.*conj(q2).*2.436924665623318e-14-q2d.*conj(q6).*7.269999999999999e+2+q3d.*conj(q5).*5.9697e+2+q4d.*conj(q4).*3.9798e+2-q5d.*conj(q3).*3.9798e+2+q6d.*conj(q2).*3.338693336175472e-14-q3d.*conj(q6).*5.4525e+2+q4d.*conj(q5).*9.9495e+2+q5d.*conj(q4).*3.9798e+2+q6d.*conj(q3).*1.8175e+2-q4d.*conj(q6).*9.0875e+2+q5d.*conj(q5).*1.59192e+3-q6d.*conj(q4).*1.8175e+2-q5d.*conj(q6).*1.454e+3-q6d.*conj(q5).*7.27e+2+q6d.*conj(q6).*3.635e+2-sqrt(3.0).*q1d.*conj(q1).*1.9899e+2-sqrt(3.0).*q1d.*conj(q2).*3.9798e+2+sqrt(3.0).*q1d.*conj(q3).*2.671400025856601e-31-sqrt(3.0).*q2d.*conj(q2).*3.9798e+2+sqrt(3.0).*q2d.*conj(q3).*2.671400025856601e-31-sqrt(3.0).*q3d.*conj(q2).*1.9899e+2-sqrt(3.0).*q1d.*conj(q5).*1.9899e+2+sqrt(3.0).*q3d.*conj(q3).*2.671400025856601e-31-sqrt(3.0).*q4d.*conj(q2).*1.9899e+2+sqrt(3.0).*q1d.*conj(q6).*1.8175e+2-sqrt(3.0).*q2d.*conj(q5).*3.9798e+2+sqrt(3.0).*q4d.*conj(q3).*1.3357000129283e-31-sqrt(3.0).*q5d.*conj(q2).*3.9798e+2+sqrt(3.0).*q2d.*conj(q6).*3.635e+2-sqrt(3.0).*q3d.*conj(q5).*1.3357000129283e-31+sqrt(3.0).*q5d.*conj(q3).*2.671400025856601e-31+sqrt(3.0).*q6d.*conj(q2).*1.8175e+2-sqrt(3.0).*q3d.*conj(q6).*2.225795557450314e-14-sqrt(3.0).*q4d.*conj(q5).*2.671400025856601e-31-sqrt(3.0).*q6d.*conj(q3).*2.225795557450315e-14-sqrt(3.0).*q4d.*conj(q6).*2.225795557450314e-14-sqrt(3.0).*q5d.*conj(q5).*5.342800051713201e-31-sqrt(3.0).*q6d.*conj(q4).*2.225795557450314e-14+sqrt(3.0).*q5d.*conj(q6).*9.75982621638147e-31+sqrt(3.0).*q6d.*conj(q5).*4.879913108190735e-31-sqrt(3.0).*q6d.*conj(q6).*4.879913108190735e-31,q1d.*(-6.047936538546912e+4)-q2d.*5.671078800000006e+3-q3d.*3.780719200000004e+3-q4d.*9.451798000000009e+3-q5d.*1.512287680000001e+4+q6d.*2.486339999999996e+3+sqrt(3.0).*q1d.*1.50919214e+4+sqrt(3.0).*q2d.*1.50919214e+4+sqrt(3.0).*q3d.*3.01838428e+4+sqrt(3.0).*q4d.*1.50919214e+4-sqrt(3.0).*q5d.*3.308806364588508e-13+sqrt(3.0).*q6d.*8.190656604720473e-14-q1d.*conj(q1).*1.218462332811659e-14-q1d.*conj(q2).*1.218462332811659e-14-q1d.*conj(q3).*3.9798e+2-q2d.*conj(q2).*1.218462332811659e-14+q1d.*conj(q4).*3.9798e+2-q2d.*conj(q3).*3.9798e+2+q1d.*conj(q5).*5.9697e+2+q2d.*conj(q4).*3.9798e+2-q3d.*conj(q3).*3.9798e+2-q1d.*conj(q6).*5.4525e+2+q2d.*conj(q5).*5.9697e+2+q3d.*conj(q4).*3.9798e+2-q4d.*conj(q3).*1.9899e+2-q2d.*conj(q6).*5.4525e+2+q3d.*conj(q5).*3.9798e+2+q4d.*conj(q4).*3.9798e+2-q5d.*conj(q3).*3.9798e+2-q3d.*conj(q6).*3.635e+2+q4d.*conj(q5).*9.9495e+2+q5d.*conj(q4).*3.9798e+2+q6d.*conj(q3).*1.8175e+2-q4d.*conj(q6).*9.0875e+2+q5d.*conj(q5).*1.59192e+3-q6d.*conj(q4).*1.8175e+2-q5d.*conj(q6).*1.454e+3-q6d.*conj(q5).*7.27e+2+q6d.*conj(q6).*3.635e+2-sqrt(3.0).*q1d.*conj(q1).*1.9899e+2-sqrt(3.0).*q1d.*conj(q2).*1.9899e+2+sqrt(3.0).*q1d.*conj(q3).*2.671400025856601e-31-sqrt(3.0).*q2d.*conj(q2).*1.9899e+2+sqrt(3.0).*q2d.*conj(q3).*2.671400025856601e-31-sqrt(3.0).*q1d.*conj(q5).*1.3357000129283e-31+sqrt(3.0).*q3d.*conj(q3).*2.671400025856601e-31-sqrt(3.0).*q1d.*conj(q6).*2.225795557450314e-14-sqrt(3.0).*q2d.*conj(q5).*1.3357000129283e-31+sqrt(3.0).*q4d.*conj(q3).*1.3357000129283e-31-sqrt(3.0).*q2d.*conj(q6).*2.225795557450314e-14+sqrt(3.0).*q5d.*conj(q3).*2.671400025856601e-31-sqrt(3.0).*q3d.*conj(q6).*4.451591114900629e-14-sqrt(3.0).*q4d.*conj(q5).*2.671400025856601e-31-sqrt(3.0).*q6d.*conj(q3).*2.225795557450315e-14-sqrt(3.0).*q4d.*conj(q6).*2.225795557450314e-14-sqrt(3.0).*q5d.*conj(q5).*5.342800051713201e-31-sqrt(3.0).*q6d.*conj(q4).*2.225795557450314e-14+sqrt(3.0).*q5d.*conj(q6).*9.75982621638147e-31+sqrt(3.0).*q6d.*conj(q5).*4.879913108190735e-31-sqrt(3.0).*q6d.*conj(q6).*4.879913108190735e-31,q1d.*(-6.426008458546913e+4)-q2d.*9.451798000000009e+3-q3d.*9.451798000000009e+3-q4d.*1.134215760000001e+4-q5d.*1.512287680000001e+4+q6d.*2.486339999999996e+3+sqrt(3.0).*q1d.*1.50919214e+4+sqrt(3.0).*q2d.*1.50919214e+4+sqrt(3.0).*q3d.*1.50919214e+4+sqrt(3.0).*q4d.*3.01838428e+4-sqrt(3.0).*q5d.*3.308806364588508e-13+sqrt(3.0).*q6d.*8.190656604720473e-14-q1d.*conj(q1).*1.218462332811659e-14-q1d.*conj(q2).*1.218462332811659e-14-q1d.*conj(q3).*1.9899e+2-q2d.*conj(q2).*1.218462332811659e-14+q1d.*conj(q4).*3.9798e+2-q2d.*conj(q3).*1.9899e+2+q1d.*conj(q5).*9.9495e+2+q2d.*conj(q4).*3.9798e+2-q3d.*conj(q3).*1.9899e+2-q1d.*conj(q6).*9.0875e+2+q2d.*conj(q5).*9.9495e+2+q3d.*conj(q4).*3.9798e+2-q2d.*conj(q6).*9.0875e+2+q3d.*conj(q5).*9.9495e+2+q4d.*conj(q4).*3.9798e+2-q3d.*conj(q6).*9.0875e+2+q4d.*conj(q5).*1.19394e+3+q5d.*conj(q4).*3.9798e+2-q4d.*conj(q6).*1.0905e+3+q5d.*conj(q5).*1.59192e+3-q6d.*conj(q4).*1.8175e+2-q5d.*conj(q6).*1.454e+3-q6d.*conj(q5).*7.27e+2+q6d.*conj(q6).*3.635e+2-sqrt(3.0).*q1d.*conj(q1).*1.9899e+2-sqrt(3.0).*q1d.*conj(q2).*1.9899e+2+sqrt(3.0).*q1d.*conj(q3).*1.3357000129283e-31-sqrt(3.0).*q2d.*conj(q2).*1.9899e+2+sqrt(3.0).*q2d.*conj(q3).*1.3357000129283e-31-sqrt(3.0).*q1d.*conj(q5).*2.671400025856601e-31+sqrt(3.0).*q3d.*conj(q3).*1.3357000129283e-31-sqrt(3.0).*q1d.*conj(q6).*2.225795557450314e-14-sqrt(3.0).*q2d.*conj(q5).*2.671400025856601e-31-sqrt(3.0).*q2d.*conj(q6).*2.225795557450314e-14-sqrt(3.0).*q3d.*conj(q5).*2.671400025856601e-31-sqrt(3.0).*q3d.*conj(q6).*2.225795557450314e-14-sqrt(3.0).*q4d.*conj(q5).*2.671400025856601e-31-sqrt(3.0).*q4d.*conj(q6).*4.451591114900629e-14-sqrt(3.0).*q5d.*conj(q5).*5.342800051713201e-31-sqrt(3.0).*q6d.*conj(q4).*2.225795557450314e-14+sqrt(3.0).*q5d.*conj(q6).*9.75982621638147e-31+sqrt(3.0).*q6d.*conj(q5).*4.879913108190735e-31-sqrt(3.0).*q6d.*conj(q6).*4.879913108190735e-31,q1d.*(-1.247394499709383e+5)-q2d.*1.512287680000001e+4-q3d.*1.512287680000001e+4-q4d.*1.512287680000001e+4-q5d.*2.268431520000002e+4-q6d.*7.320196429342594e-12+sqrt(3.0).*q1d.*6.381198636905707e-12-sqrt(3.0).*q2d.*3.308806364588508e-13-sqrt(3.0).*q3d.*3.308806364588508e-13-sqrt(3.0).*q4d.*3.308806364588508e-13-sqrt(3.0).*q5d.*4.963209546882762e-13-sqrt(3.0).*q6d.*1.668930283001236e-30-q1d.*conj(q1).*2.436924665623318e-14-q1d.*conj(q2).*2.436924665623318e-14-q1d.*conj(q3).*3.9798e+2-q2d.*conj(q2).*2.436924665623318e-14+q1d.*conj(q4).*3.9798e+2-q2d.*conj(q3).*3.9798e+2+q1d.*conj(q5).*1.59192e+3+q2d.*conj(q4).*3.9798e+2-q3d.*conj(q3).*3.9798e+2-q1d.*conj(q6).*1.454e+3+q2d.*conj(q5).*1.59192e+3+q3d.*conj(q4).*3.9798e+2-q2d.*conj(q6).*1.454e+3+q3d.*conj(q5).*1.59192e+3+q4d.*conj(q4).*3.9798e+2-q3d.*conj(q6).*1.454e+3+q4d.*conj(q5).*1.59192e+3-q4d.*conj(q6).*1.454e+3+q5d.*conj(q5).*2.38788e+3-q5d.*conj(q6).*2.181e+3-q6d.*conj(q5).*7.27e+2+q6d.*conj(q6).*1.090325361995171e-29-sqrt(3.0).*q1d.*conj(q1).*3.9798e+2-sqrt(3.0).*q1d.*conj(q2).*3.9798e+2+sqrt(3.0).*q1d.*conj(q3).*2.671400025856601e-31-sqrt(3.0).*q2d.*conj(q2).*3.9798e+2+sqrt(3.0).*q2d.*conj(q3).*2.671400025856601e-31-sqrt(3.0).*q1d.*conj(q5).*5.342800051713201e-31+sqrt(3.0).*q3d.*conj(q3).*2.671400025856601e-31+sqrt(3.0).*q1d.*conj(q6).*9.75982621638147e-31-sqrt(3.0).*q2d.*conj(q5).*5.342800051713201e-31+sqrt(3.0).*q2d.*conj(q6).*9.75982621638147e-31-sqrt(3.0).*q3d.*conj(q5).*5.342800051713201e-31+sqrt(3.0).*q3d.*conj(q6).*9.75982621638147e-31-sqrt(3.0).*q4d.*conj(q5).*5.342800051713201e-31+sqrt(3.0).*q4d.*conj(q6).*9.75982621638147e-31-sqrt(3.0).*q5d.*conj(q5).*8.014200077569802e-31+sqrt(3.0).*q5d.*conj(q6).*1.46397393245722e-30+sqrt(3.0).*q6d.*conj(q5).*4.879913108190735e-31-sqrt(3.0).*q6d.*conj(q6).*2.439956554095367e-31,q1d.*5.254617258912011e+4+q2d.*2.486339999999996e+3+q3d.*2.486339999999996e+3+q4d.*2.486339999999996e+3-q5d.*7.320196429342594e-12+q6d.*9.94536e+3-sqrt(3.0).*q1d.*9.113935495870542e-12+sqrt(3.0).*q2d.*8.190656604720473e-14+sqrt(3.0).*q3d.*8.190656604720473e-14+sqrt(3.0).*q4d.*8.190656604720473e-14-sqrt(3.0).*q5d.*1.668930283001236e-30+sqrt(3.0).*q6d.*3.276262641888189e-13+q1d.*conj(q1).*3.338693336175472e-14+q1d.*conj(q2).*3.338693336175472e-14+q1d.*conj(q3).*1.8175e+2+q2d.*conj(q2).*3.338693336175472e-14-q1d.*conj(q4).*1.8175e+2+q2d.*conj(q3).*1.8175e+2-q1d.*conj(q5).*7.27e+2-q2d.*conj(q4).*1.8175e+2+q3d.*conj(q3).*1.8175e+2+q1d.*conj(q6).*3.635e+2-q2d.*conj(q5).*7.27e+2-q3d.*conj(q4).*1.8175e+2+q2d.*conj(q6).*3.635e+2-q3d.*conj(q5).*7.27e+2-q4d.*conj(q4).*1.8175e+2+q3d.*conj(q6).*3.635e+2-q4d.*conj(q5).*7.27e+2+q4d.*conj(q6).*3.635e+2-q5d.*conj(q5).*7.27e+2+q5d.*conj(q6).*1.090325361995171e-29-q6d.*conj(q5).*7.27e+2+q6d.*conj(q6).*1.454e+3+sqrt(3.0).*q1d.*conj(q1).*1.8175e+2+sqrt(3.0).*q1d.*conj(q2).*1.8175e+2-sqrt(3.0).*q1d.*conj(q3).*2.225795557450315e-14+sqrt(3.0).*q2d.*conj(q2).*1.8175e+2-sqrt(3.0).*q1d.*conj(q4).*2.225795557450314e-14-sqrt(3.0).*q2d.*conj(q3).*2.225795557450315e-14+sqrt(3.0).*q1d.*conj(q5).*4.879913108190735e-31-sqrt(3.0).*q2d.*conj(q4).*2.225795557450314e-14-sqrt(3.0).*q3d.*conj(q3).*2.225795557450315e-14-sqrt(3.0).*q1d.*conj(q6).*4.879913108190735e-31+sqrt(3.0).*q2d.*conj(q5).*4.879913108190735e-31-sqrt(3.0).*q3d.*conj(q4).*2.225795557450314e-14-sqrt(3.0).*q2d.*conj(q6).*4.879913108190735e-31+sqrt(3.0).*q3d.*conj(q5).*4.879913108190735e-31-sqrt(3.0).*q4d.*conj(q4).*2.225795557450314e-14-sqrt(3.0).*q3d.*conj(q6).*4.879913108190735e-31+sqrt(3.0).*q4d.*conj(q5).*4.879913108190735e-31-sqrt(3.0).*q4d.*conj(q6).*4.879913108190735e-31+sqrt(3.0).*q5d.*conj(q5).*4.879913108190735e-31-sqrt(3.0).*q5d.*conj(q6).*2.439956554095367e-31+sqrt(3.0).*q6d.*conj(q5).*4.879913108190735e-31-sqrt(3.0).*q6d.*conj(q6).*1.46397393245722e-30,q1d.*7.520537517824024e+4+q2d.*4.008902758912012e+4+q3d.*5.627568258912012e+4+q4d.*5.378934258912012e+4+q5d.*5.254617258912011e+4+q6d.*1.100650251782402e+5+sqrt(3.0).*q1d.*2.486339999999987e+3+sqrt(3.0).*q2d.*1.243169999999994e+3+sqrt(3.0).*q3d.*1.494348499999999e+4+sqrt(3.0).*q4d.*1.494348499999999e+4-sqrt(3.0).*q5d.*9.113935495870542e-12-sqrt(3.0).*q6d.*1.806405785964667e-11+q1d.*conj(q1).*6.677386672350943e-14+q1d.*conj(q2).*6.677386672350943e-14+q2d.*conj(q1).*3.338693336175472e-14+q1d.*conj(q3).*3.635e+2+q2d.*conj(q2).*6.677386672350943e-14+q3d.*conj(q1).*3.338693336175472e-14-q1d.*conj(q4).*3.635e+2+q2d.*conj(q3).*3.635e+2+q3d.*conj(q2).*3.338693336175472e-14+q4d.*conj(q1).*3.338693336175472e-14-q1d.*conj(q5).*7.27e+2-q2d.*conj(q4).*3.635e+2+q3d.*conj(q3).*3.635e+2+q4d.*conj(q2).*3.338693336175472e-14+q5d.*conj(q1).*3.338693336175472e-14+q1d.*conj(q6).*7.270000000000001e+2-q2d.*conj(q5).*7.27e+2-q3d.*conj(q4).*3.635e+2+q4d.*conj(q3).*1.8175e+2+q5d.*conj(q2).*3.338693336175472e-14+q6d.*conj(q1).*6.677386672350943e-14+q2d.*conj(q6).*7.27e+2-q3d.*conj(q5).*7.27e+2-q4d.*conj(q4).*3.635e+2+q5d.*conj(q3).*1.8175e+2+q6d.*conj(q2).*6.677386672350943e-14+q3d.*conj(q6).*9.0875e+2-q4d.*conj(q5).*7.27e+2-q5d.*conj(q4).*1.8175e+2+q6d.*conj(q3).*3.635e+2+q4d.*conj(q6).*5.4525e+2-q5d.*conj(q5).*7.27e+2-q6d.*conj(q4).*3.635e+2+q5d.*conj(q6).*3.635e+2-q6d.*conj(q5).*7.27e+2+q6d.*conj(q6).*1.454e+3+sqrt(3.0).*q1d.*conj(q1).*3.635e+2+sqrt(3.0).*q1d.*conj(q2).*3.635e+2+sqrt(3.0).*q2d.*conj(q1).*1.8175e+2-sqrt(3.0).*q1d.*conj(q3).*4.451591114900629e-14+sqrt(3.0).*q2d.*conj(q2).*3.635e+2+sqrt(3.0).*q3d.*conj(q1).*1.8175e+2-sqrt(3.0).*q1d.*conj(q4).*4.451591114900629e-14-sqrt(3.0).*q2d.*conj(q3).*4.451591114900629e-14+sqrt(3.0).*q3d.*conj(q2).*1.8175e+2+sqrt(3.0).*q4d.*conj(q1).*1.8175e+2+sqrt(3.0).*q1d.*conj(q5).*4.879913108190735e-31-sqrt(3.0).*q2d.*conj(q4).*4.451591114900629e-14-sqrt(3.0).*q3d.*conj(q3).*4.451591114900629e-14+sqrt(3.0).*q4d.*conj(q2).*1.8175e+2+sqrt(3.0).*q5d.*conj(q1).*1.8175e+2+sqrt(3.0).*q1d.*conj(q6).*3.635e+2+sqrt(3.0).*q2d.*conj(q5).*4.879913108190735e-31-sqrt(3.0).*q3d.*conj(q4).*4.451591114900629e-14-sqrt(3.0).*q4d.*conj(q3).*2.225795557450315e-14+sqrt(3.0).*q5d.*conj(q2).*1.8175e+2+sqrt(3.0).*q6d.*conj(q1).*3.635e+2+sqrt(3.0).*q2d.*conj(q6).*1.8175e+2+sqrt(3.0).*q3d.*conj(q5).*4.879913108190735e-31-sqrt(3.0).*q4d.*conj(q4).*4.451591114900629e-14-sqrt(3.0).*q5d.*conj(q3).*2.225795557450315e-14+sqrt(3.0).*q6d.*conj(q2).*3.635e+2-sqrt(3.0).*q3d.*conj(q6).*2.225795557450315e-14+sqrt(3.0).*q4d.*conj(q5).*4.879913108190735e-31-sqrt(3.0).*q5d.*conj(q4).*2.225795557450314e-14-sqrt(3.0).*q6d.*conj(q3).*4.451591114900629e-14-sqrt(3.0).*q4d.*conj(q6).*2.225795557450315e-14+sqrt(3.0).*q5d.*conj(q5).*4.879913108190735e-31-sqrt(3.0).*q6d.*conj(q4).*4.451591114900629e-14-sqrt(3.0).*q5d.*conj(q6).*4.879913108190735e-31+sqrt(3.0).*q6d.*conj(q5).*4.879913108190735e-31-sqrt(3.0).*q6d.*conj(q6).*1.46397393245722e-30,q1d.*4.008902758912012e+4-q2d.*2.491429e+4+q3d.*6.215850000000002e+3+q4d.*3.729509999999998e+3+q5d.*2.486339999999996e+3+q6d.*9.94536e+3+sqrt(3.0).*q1d.*1.243169999999994e+3+sqrt(3.0).*q2d.*2.486340000000006e+3+sqrt(3.0).*q3d.*1.4943485e+4+sqrt(3.0).*q4d.*1.4943485e+4+sqrt(3.0).*q5d.*8.190656604720473e-14+sqrt(3.0).*q6d.*3.276262641888189e-13+q1d.*conj(q1).*3.338693336175472e-14+q1d.*conj(q2).*6.677386672350943e-14+q1d.*conj(q3).*3.635e+2+q2d.*conj(q2).*6.677386672350943e-14-q1d.*conj(q4).*3.635e+2+q2d.*conj(q3).*3.635e+2+q3d.*conj(q2).*3.338693336175472e-14-q1d.*conj(q5).*7.27e+2-q2d.*conj(q4).*3.635e+2+q3d.*conj(q3).*3.635e+2+q4d.*conj(q2).*3.338693336175472e-14+q1d.*conj(q6).*7.27e+2-q2d.*conj(q5).*7.27e+2-q3d.*conj(q4).*3.635e+2+q4d.*conj(q3).*1.8175e+2+q5d.*conj(q2).*3.338693336175472e-14+q2d.*conj(q6).*7.270000000000001e+2-q3d.*conj(q5).*7.27e+2-q4d.*conj(q4).*3.635e+2+q5d.*conj(q3).*1.8175e+2+q6d.*conj(q2).*6.677386672350943e-14+q3d.*conj(q6).*9.0875e+2-q4d.*conj(q5).*7.27e+2-q5d.*conj(q4).*1.8175e+2+q6d.*conj(q3).*3.635e+2+q4d.*conj(q6).*5.4525e+2-q5d.*conj(q5).*7.27e+2-q6d.*conj(q4).*3.635e+2+q5d.*conj(q6).*3.635e+2-q6d.*conj(q5).*7.27e+2+q6d.*conj(q6).*1.454e+3+sqrt(3.0).*q1d.*conj(q1).*1.8175e+2+sqrt(3.0).*q1d.*conj(q2).*3.635e+2-sqrt(3.0).*q1d.*conj(q3).*4.451591114900629e-14+sqrt(3.0).*q2d.*conj(q2).*3.635e+2-sqrt(3.0).*q1d.*conj(q4).*4.451591114900629e-14-sqrt(3.0).*q2d.*conj(q3).*4.451591114900629e-14+sqrt(3.0).*q3d.*conj(q2).*1.8175e+2+sqrt(3.0).*q1d.*conj(q5).*4.879913108190735e-31-sqrt(3.0).*q2d.*conj(q4).*4.451591114900629e-14-sqrt(3.0).*q3d.*conj(q3).*4.451591114900629e-14+sqrt(3.0).*q4d.*conj(q2).*1.8175e+2+sqrt(3.0).*q1d.*conj(q6).*1.8175e+2+sqrt(3.0).*q2d.*conj(q5).*4.879913108190735e-31-sqrt(3.0).*q3d.*conj(q4).*4.451591114900629e-14-sqrt(3.0).*q4d.*conj(q3).*2.225795557450315e-14+sqrt(3.0).*q5d.*conj(q2).*1.8175e+2+sqrt(3.0).*q2d.*conj(q6).*3.635e+2+sqrt(3.0).*q3d.*conj(q5).*4.879913108190735e-31-sqrt(3.0).*q4d.*conj(q4).*4.451591114900629e-14-sqrt(3.0).*q5d.*conj(q3).*2.225795557450315e-14+sqrt(3.0).*q6d.*conj(q2).*3.635e+2-sqrt(3.0).*q3d.*conj(q6).*2.225795557450315e-14+sqrt(3.0).*q4d.*conj(q5).*4.879913108190735e-31-sqrt(3.0).*q5d.*conj(q4).*2.225795557450314e-14-sqrt(3.0).*q6d.*conj(q3).*4.451591114900629e-14-sqrt(3.0).*q4d.*conj(q6).*2.225795557450315e-14+sqrt(3.0).*q5d.*conj(q5).*4.879913108190735e-31-sqrt(3.0).*q6d.*conj(q4).*4.451591114900629e-14-sqrt(3.0).*q5d.*conj(q6).*4.879913108190735e-31+sqrt(3.0).*q6d.*conj(q5).*4.879913108190735e-31-sqrt(3.0).*q6d.*conj(q6).*1.46397393245722e-30,q1d.*5.627568258912012e+4+q2d.*6.215850000000002e+3+q3d.*7.459020000000004e+3+q4d.*3.729509999999998e+3+q5d.*2.486339999999996e+3+q6d.*9.94536e+3+sqrt(3.0).*q1d.*1.494348499999999e+4+sqrt(3.0).*q2d.*1.4943485e+4+sqrt(3.0).*q3d.*2.988697e+4+sqrt(3.0).*q4d.*1.4943485e+4+sqrt(3.0).*q5d.*8.190656604720473e-14+sqrt(3.0).*q6d.*3.276262641888189e-13+q1d.*conj(q1).*3.338693336175472e-14+q1d.*conj(q2).*3.338693336175472e-14+q1d.*conj(q3).*3.635e+2+q2d.*conj(q2).*3.338693336175472e-14-q1d.*conj(q4).*3.635e+2+q2d.*conj(q3).*3.635e+2-q1d.*conj(q5).*7.27e+2-q2d.*conj(q4).*3.635e+2+q3d.*conj(q3).*3.635e+2+q1d.*conj(q6).*9.0875e+2-q2d.*conj(q5).*7.27e+2-q3d.*conj(q4).*3.635e+2+q4d.*conj(q3).*1.8175e+2+q2d.*conj(q6).*9.0875e+2-q3d.*conj(q5).*7.27e+2-q4d.*conj(q4).*3.635e+2+q5d.*conj(q3).*1.8175e+2+q3d.*conj(q6).*1.0905e+3-q4d.*conj(q5).*7.27e+2-q5d.*conj(q4).*1.8175e+2+q6d.*conj(q3).*3.635e+2+q4d.*conj(q6).*5.4525e+2-q5d.*conj(q5).*7.27e+2-q6d.*conj(q4).*3.635e+2+q5d.*conj(q6).*3.635e+2-q6d.*conj(q5).*7.27e+2+q6d.*conj(q6).*1.454e+3+sqrt(3.0).*q1d.*conj(q1).*1.8175e+2+sqrt(3.0).*q1d.*conj(q2).*1.8175e+2-sqrt(3.0).*q1d.*conj(q3).*4.451591114900629e-14+sqrt(3.0).*q2d.*conj(q2).*1.8175e+2-sqrt(3.0).*q1d.*conj(q4).*4.451591114900629e-14-sqrt(3.0).*q2d.*conj(q3).*4.451591114900629e-14+sqrt(3.0).*q1d.*conj(q5).*4.879913108190735e-31-sqrt(3.0).*q2d.*conj(q4).*4.451591114900629e-14-sqrt(3.0).*q3d.*conj(q3).*4.451591114900629e-14-sqrt(3.0).*q1d.*conj(q6).*2.225795557450315e-14+sqrt(3.0).*q2d.*conj(q5).*4.879913108190735e-31-sqrt(3.0).*q3d.*conj(q4).*4.451591114900629e-14-sqrt(3.0).*q4d.*conj(q3).*2.225795557450315e-14-sqrt(3.0).*q2d.*conj(q6).*2.225795557450315e-14+sqrt(3.0).*q3d.*conj(q5).*4.879913108190735e-31-sqrt(3.0).*q4d.*conj(q4).*4.451591114900629e-14-sqrt(3.0).*q5d.*conj(q3).*2.225795557450315e-14-sqrt(3.0).*q3d.*conj(q6).*4.451591114900629e-14+sqrt(3.0).*q4d.*conj(q5).*4.879913108190735e-31-sqrt(3.0).*q5d.*conj(q4).*2.225795557450314e-14-sqrt(3.0).*q6d.*conj(q3).*4.451591114900629e-14-sqrt(3.0).*q4d.*conj(q6).*2.225795557450315e-14+sqrt(3.0).*q5d.*conj(q5).*4.879913108190735e-31-sqrt(3.0).*q6d.*conj(q4).*4.451591114900629e-14-sqrt(3.0).*q5d.*conj(q6).*4.879913108190735e-31+sqrt(3.0).*q6d.*conj(q5).*4.879913108190735e-31-sqrt(3.0).*q6d.*conj(q6).*1.46397393245722e-30,q1d.*5.378934258912012e+4+q2d.*3.729509999999998e+3+q3d.*3.729509999999998e+3+q4d.*2.486339999999996e+3+q5d.*2.486339999999996e+3+q6d.*9.94536e+3+sqrt(3.0).*q1d.*1.494348499999999e+4+sqrt(3.0).*q2d.*1.4943485e+4+sqrt(3.0).*q3d.*1.4943485e+4+sqrt(3.0).*q4d.*2.988697e+4+sqrt(3.0).*q5d.*8.190656604720473e-14+sqrt(3.0).*q6d.*3.276262641888189e-13+q1d.*conj(q1).*3.338693336175472e-14+q1d.*conj(q2).*3.338693336175472e-14+q1d.*conj(q3).*1.8175e+2+q2d.*conj(q2).*3.338693336175472e-14-q1d.*conj(q4).*3.635e+2+q2d.*conj(q3).*1.8175e+2-q1d.*conj(q5).*7.27e+2-q2d.*conj(q4).*3.635e+2+q3d.*conj(q3).*1.8175e+2+q1d.*conj(q6).*5.4525e+2-q2d.*conj(q5).*7.27e+2-q3d.*conj(q4).*3.635e+2+q2d.*conj(q6).*5.4525e+2-q3d.*conj(q5).*7.27e+2-q4d.*conj(q4).*3.635e+2+q3d.*conj(q6).*5.4525e+2-q4d.*conj(q5).*7.27e+2-q5d.*conj(q4).*1.8175e+2+q4d.*conj(q6).*3.635e+2-q5d.*conj(q5).*7.27e+2-q6d.*conj(q4).*3.635e+2+q5d.*conj(q6).*3.635e+2-q6d.*conj(q5).*7.27e+2+q6d.*conj(q6).*1.454e+3+sqrt(3.0).*q1d.*conj(q1).*1.8175e+2+sqrt(3.0).*q1d.*conj(q2).*1.8175e+2-sqrt(3.0).*q1d.*conj(q3).*2.225795557450315e-14+sqrt(3.0).*q2d.*conj(q2).*1.8175e+2-sqrt(3.0).*q1d.*conj(q4).*4.451591114900629e-14-sqrt(3.0).*q2d.*conj(q3).*2.225795557450315e-14+sqrt(3.0).*q1d.*conj(q5).*4.879913108190735e-31-sqrt(3.0).*q2d.*conj(q4).*4.451591114900629e-14-sqrt(3.0).*q3d.*conj(q3).*2.225795557450315e-14-sqrt(3.0).*q1d.*conj(q6).*2.225795557450315e-14+sqrt(3.0).*q2d.*conj(q5).*4.879913108190735e-31-sqrt(3.0).*q3d.*conj(q4).*4.451591114900629e-14-sqrt(3.0).*q2d.*conj(q6).*2.225795557450315e-14+sqrt(3.0).*q3d.*conj(q5).*4.879913108190735e-31-sqrt(3.0).*q4d.*conj(q4).*4.451591114900629e-14-sqrt(3.0).*q3d.*conj(q6).*2.225795557450315e-14+sqrt(3.0).*q4d.*conj(q5).*4.879913108190735e-31-sqrt(3.0).*q5d.*conj(q4).*2.225795557450314e-14-sqrt(3.0).*q4d.*conj(q6).*4.451591114900629e-14+sqrt(3.0).*q5d.*conj(q5).*4.879913108190735e-31-sqrt(3.0).*q6d.*conj(q4).*4.451591114900629e-14-sqrt(3.0).*q5d.*conj(q6).*4.879913108190735e-31+sqrt(3.0).*q6d.*conj(q5).*4.879913108190735e-31-sqrt(3.0).*q6d.*conj(q6).*1.46397393245722e-30,q1d.*5.254617258912011e+4+q2d.*2.486339999999996e+3+q3d.*2.486339999999996e+3+q4d.*2.486339999999996e+3-q5d.*7.320196429342594e-12+q6d.*9.94536e+3-sqrt(3.0).*q1d.*9.113935495870542e-12+sqrt(3.0).*q2d.*8.190656604720473e-14+sqrt(3.0).*q3d.*8.190656604720473e-14+sqrt(3.0).*q4d.*8.190656604720473e-14-sqrt(3.0).*q5d.*1.668930283001236e-30+sqrt(3.0).*q6d.*3.276262641888189e-13+q1d.*conj(q1).*3.338693336175472e-14+q1d.*conj(q2).*3.338693336175472e-14+q1d.*conj(q3).*1.8175e+2+q2d.*conj(q2).*3.338693336175472e-14-q1d.*conj(q4).*1.8175e+2+q2d.*conj(q3).*1.8175e+2-q1d.*conj(q5).*7.27e+2-q2d.*conj(q4).*1.8175e+2+q3d.*conj(q3).*1.8175e+2+q1d.*conj(q6).*3.635e+2-q2d.*conj(q5).*7.27e+2-q3d.*conj(q4).*1.8175e+2+q2d.*conj(q6).*3.635e+2-q3d.*conj(q5).*7.27e+2-q4d.*conj(q4).*1.8175e+2+q3d.*conj(q6).*3.635e+2-q4d.*conj(q5).*7.27e+2+q4d.*conj(q6).*3.635e+2-q5d.*conj(q5).*7.27e+2+q5d.*conj(q6).*1.090325361995171e-29-q6d.*conj(q5).*7.27e+2+q6d.*conj(q6).*1.454e+3+sqrt(3.0).*q1d.*conj(q1).*1.8175e+2+sqrt(3.0).*q1d.*conj(q2).*1.8175e+2-sqrt(3.0).*q1d.*conj(q3).*2.225795557450315e-14+sqrt(3.0).*q2d.*conj(q2).*1.8175e+2-sqrt(3.0).*q1d.*conj(q4).*2.225795557450314e-14-sqrt(3.0).*q2d.*conj(q3).*2.225795557450315e-14+sqrt(3.0).*q1d.*conj(q5).*4.879913108190735e-31-sqrt(3.0).*q2d.*conj(q4).*2.225795557450314e-14-sqrt(3.0).*q3d.*conj(q3).*2.225795557450315e-14-sqrt(3.0).*q1d.*conj(q6).*4.879913108190735e-31+sqrt(3.0).*q2d.*conj(q5).*4.879913108190735e-31-sqrt(3.0).*q3d.*conj(q4).*2.225795557450314e-14-sqrt(3.0).*q2d.*conj(q6).*4.879913108190735e-31+sqrt(3.0).*q3d.*conj(q5).*4.879913108190735e-31-sqrt(3.0).*q4d.*conj(q4).*2.225795557450314e-14-sqrt(3.0).*q3d.*conj(q6).*4.879913108190735e-31+sqrt(3.0).*q4d.*conj(q5).*4.879913108190735e-31-sqrt(3.0).*q4d.*conj(q6).*4.879913108190735e-31+sqrt(3.0).*q5d.*conj(q5).*4.879913108190735e-31-sqrt(3.0).*q5d.*conj(q6).*2.439956554095367e-31+sqrt(3.0).*q6d.*conj(q5).*4.879913108190735e-31-sqrt(3.0).*q6d.*conj(q6).*1.46397393245722e-30,q1d.*1.100650251782402e+5+q2d.*9.94536e+3+q3d.*9.94536e+3+q4d.*9.94536e+3+q5d.*9.94536e+3+q6d.*1.491804e+4-sqrt(3.0).*q1d.*1.806405785964667e-11+sqrt(3.0).*q2d.*3.276262641888189e-13+sqrt(3.0).*q3d.*3.276262641888189e-13+sqrt(3.0).*q4d.*3.276262641888189e-13+sqrt(3.0).*q5d.*3.276262641888189e-13+sqrt(3.0).*q6d.*4.914393962832284e-13+q1d.*conj(q1).*6.677386672350943e-14+q1d.*conj(q2).*6.677386672350943e-14+q1d.*conj(q3).*3.635e+2+q2d.*conj(q2).*6.677386672350943e-14-q1d.*conj(q4).*3.635e+2+q2d.*conj(q3).*3.635e+2-q1d.*conj(q5).*7.27e+2-q2d.*conj(q4).*3.635e+2+q3d.*conj(q3).*3.635e+2+q1d.*conj(q6).*1.454e+3-q2d.*conj(q5).*7.27e+2-q3d.*conj(q4).*3.635e+2+q2d.*conj(q6).*1.454e+3-q3d.*conj(q5).*7.27e+2-q4d.*conj(q4).*3.635e+2+q3d.*conj(q6).*1.454e+3-q4d.*conj(q5).*7.27e+2+q4d.*conj(q6).*1.454e+3-q5d.*conj(q5).*7.27e+2+q5d.*conj(q6).*1.454e+3+q6d.*conj(q6).*2.181e+3+sqrt(3.0).*q1d.*conj(q1).*3.635e+2+sqrt(3.0).*q1d.*conj(q2).*3.635e+2-sqrt(3.0).*q1d.*conj(q3).*4.451591114900629e-14+sqrt(3.0).*q2d.*conj(q2).*3.635e+2-sqrt(3.0).*q1d.*conj(q4).*4.451591114900629e-14-sqrt(3.0).*q2d.*conj(q3).*4.451591114900629e-14+sqrt(3.0).*q1d.*conj(q5).*4.879913108190735e-31-sqrt(3.0).*q2d.*conj(q4).*4.451591114900629e-14-sqrt(3.0).*q3d.*conj(q3).*4.451591114900629e-14-sqrt(3.0).*q1d.*conj(q6).*1.46397393245722e-30+sqrt(3.0).*q2d.*conj(q5).*4.879913108190735e-31-sqrt(3.0).*q3d.*conj(q4).*4.451591114900629e-14-sqrt(3.0).*q2d.*conj(q6).*1.46397393245722e-30+sqrt(3.0).*q3d.*conj(q5).*4.879913108190735e-31-sqrt(3.0).*q4d.*conj(q4).*4.451591114900629e-14-sqrt(3.0).*q3d.*conj(q6).*1.46397393245722e-30+sqrt(3.0).*q4d.*conj(q5).*4.879913108190735e-31-sqrt(3.0).*q4d.*conj(q6).*1.46397393245722e-30+sqrt(3.0).*q5d.*conj(q5).*4.879913108190735e-31-sqrt(3.0).*q5d.*conj(q6).*1.46397393245722e-30-sqrt(3.0).*q6d.*conj(q6).*2.195960898685831e-30],[6,6]);


%%%%%%%%%%%%%%%%%%%%%%%
